simulink model "CVS Model"  (R2021a)
(part 5 of 8)

  R-Rdial Artery4 : ee_lib/Passive/Resistor  R=19.139 kOhm  R_tol=5  enable_R_tol=0  tol_distribution=1  nSigma=4  enable_operating_limits=0  operating_limit_action=2  max_working_voltage=100 V  power_rating=1 W  enable_faults=0  fault_action=1  R_faulted=inf Ohm  enable_temporal_fault=0  t_fault=1 s  enable_behavioral_fault=0  max_permissible_current=1 A  t_fail_on_current=1 s  noise_mode=0  sample_time=1e-3 s  repeatability=1  auto_seed=1105989530  user_seed=0  Tdevice=25 degC  alpha=3.93e-3 1/K  Tmeas=25 degC  thermal_mass=100 J/K  power_derating_T1=70 degC  power_derating_T2=155 degC  operating_temperature_range_vec=[-50, 150] degC  temperature_specify=off  temperature_priority=High  temperature=298.15 K  temperature_nominal_specify=off  temperature_nominal_unit=K  temperature_nominal_value=1
  R-Rdial Artery5 : ee_lib/Passive/Resistor  R=11 kOhm  R_tol=5  enable_R_tol=0  tol_distribution=1  nSigma=4  enable_operating_limits=0  operating_limit_action=2  max_working_voltage=100 V  power_rating=1 W  enable_faults=0  fault_action=1  R_faulted=inf Ohm  enable_temporal_fault=0  t_fault=1 s  enable_behavioral_fault=0  max_permissible_current=1 A  t_fail_on_current=1 s  noise_mode=0  sample_time=1e-3 s  repeatability=1  auto_seed=3610853119  user_seed=0  Tdevice=25 degC  alpha=3.93e-3 1/K  Tmeas=25 degC  thermal_mass=100 J/K  power_derating_T1=70 degC  power_derating_T2=155 degC  operating_temperature_range_vec=[-50, 150] degC  temperature_specify=off  temperature_priority=High  temperature=298.15 K  temperature_nominal_specify=off  temperature_nominal_unit=K  temperature_nominal_value=1
  R-Rdial Artery6 : ee_lib/Passive/Resistor  Commented=on  R=19.139 kOhm  R_tol=5  enable_R_tol=0  tol_distribution=1  nSigma=4  enable_operating_limits=0  operating_limit_action=2  max_working_voltage=100 V  power_rating=1 W  enable_faults=0  fault_action=1  R_faulted=inf Ohm  enable_temporal_fault=0  t_fault=1 s  enable_behavioral_fault=0  max_permissible_current=1 A  t_fail_on_current=1 s  noise_mode=0  sample_time=1e-3 s  repeatability=1  auto_seed=2563070851  user_seed=0  Tdevice=25 degC  alpha=3.93e-3 1/K  Tmeas=25 degC  thermal_mass=100 J/K  power_derating_T1=70 degC  power_derating_T2=155 degC  operating_temperature_range_vec=[-50, 150] degC  temperature_specify=off  temperature_priority=High  temperature=298.15 K  temperature_nominal_specify=off  temperature_nominal_unit=K  temperature_nominal_value=1
  R-Rdial Artery7 : ee_lib/Passive/Resistor  Commented=on  R=11 kOhm  R_tol=5  enable_R_tol=0  tol_distribution=1  nSigma=4  enable_operating_limits=0  operating_limit_action=2  max_working_voltage=100 V  power_rating=1 W  enable_faults=0  fault_action=1  R_faulted=inf Ohm  enable_temporal_fault=0  t_fault=1 s  enable_behavioral_fault=0  max_permissible_current=1 A  t_fail_on_current=1 s  noise_mode=0  sample_time=1e-3 s  repeatability=1  auto_seed=2518122460  user_seed=0  Tdevice=25 degC  alpha=3.93e-3 1/K  Tmeas=25 degC  thermal_mass=100 J/K  power_derating_T1=70 degC  power_derating_T2=155 degC  operating_temperature_range_vec=[-50, 150] degC  temperature_specify=off  temperature_priority=High  temperature=298.15 K  temperature_nominal_specify=off  temperature_nominal_unit=K  temperature_nominal_value=1
  R-Rdial Artery8 : ee_lib/Passive/Resistor  R=19.139 kOhm  R_tol=5  enable_R_tol=0  tol_distribution=1  nSigma=4  enable_operating_limits=0  operating_limit_action=2  max_working_voltage=100 V  power_rating=1 W  enable_faults=0  fault_action=1  R_faulted=inf Ohm  enable_temporal_fault=0  t_fault=1 s  enable_behavioral_fault=0  max_permissible_current=1 A  t_fail_on_current=1 s  noise_mode=0  sample_time=1e-3 s  repeatability=1  auto_seed=1105989530  user_seed=0  Tdevice=25 degC  alpha=3.93e-3 1/K  Tmeas=25 degC  thermal_mass=100 J/K  power_derating_T1=70 degC  power_derating_T2=155 degC  operating_temperature_range_vec=[-50, 150] degC  temperature_specify=off  temperature_priority=High  temperature=298.15 K  temperature_nominal_specify=off  temperature_nominal_unit=K  temperature_nominal_value=1
  R-Rdial Artery9 : ee_lib/Passive/Resistor  R=11 kOhm  R_tol=5  enable_R_tol=0  tol_distribution=1  nSigma=4  enable_operating_limits=0  operating_limit_action=2  max_working_voltage=100 V  power_rating=1 W  enable_faults=0  fault_action=1  R_faulted=inf Ohm  enable_temporal_fault=0  t_fault=1 s  enable_behavioral_fault=0  max_permissible_current=1 A  t_fail_on_current=1 s  noise_mode=0  sample_time=1e-3 s  repeatability=1  auto_seed=3610853119  user_seed=0  Tdevice=25 degC  alpha=3.93e-3 1/K  Tmeas=25 degC  thermal_mass=100 J/K  power_derating_T1=70 degC  power_derating_T2=155 degC  operating_temperature_range_vec=[-50, 150] degC  temperature_specify=off  temperature_priority=High  temperature=298.15 K  temperature_nominal_specify=off  temperature_nominal_unit=K  temperature_nominal_value=1
  R-Right Common Iliac1 : ee_lib/Passive/Resistor  Commented=on  R=0.43 kOhm  R_tol=5  enable_R_tol=0  tol_distribution=1  nSigma=4  enable_operating_limits=0  operating_limit_action=2  max_working_voltage=100 V  power_rating=1 W  enable_faults=0  fault_action=1  R_faulted=inf Ohm  enable_temporal_fault=0  t_fault=1 s  enable_behavioral_fault=0  max_permissible_current=1 A  t_fail_on_current=1 s  noise_mode=0  sample_time=1e-3 s  repeatability=1  auto_seed=1147740212  user_seed=0  Tdevice=25 degC  alpha=3.93e-3 1/K  Tmeas=25 degC  thermal_mass=100 J/K  power_derating_T1=70 degC  power_derating_T2=155 degC  operating_temperature_range_vec=[-50, 150] degC  temperature_specify=off  temperature_priority=High  temperature=298.15 K  temperature_nominal_specify=off  temperature_nominal_unit=K  temperature_nominal_value=1
  R-Right Common Iliac2 : ee_lib/Passive/Resistor  R=0.43 kOhm  R_tol=5  enable_R_tol=0  tol_distribution=1  nSigma=4  enable_operating_limits=0  operating_limit_action=2  max_working_voltage=100 V  power_rating=1 W  enable_faults=0  fault_action=1  R_faulted=inf Ohm  enable_temporal_fault=0  t_fault=1 s  enable_behavioral_fault=0  max_permissible_current=1 A  t_fail_on_current=1 s  noise_mode=0  sample_time=1e-3 s  repeatability=1  auto_seed=1092133643  user_seed=0  Tdevice=25 degC  alpha=3.93e-3 1/K  Tmeas=25 degC  thermal_mass=100 J/K  power_derating_T1=70 degC  power_derating_T2=155 degC  operating_temperature_range_vec=[-50, 150] degC  temperature_specify=off  temperature_priority=High  temperature=298.15 K  temperature_nominal_specify=off  temperature_nominal_unit=K  temperature_nominal_value=1
  R-Right Common Iliac3 : ee_lib/Passive/Resistor  Commented=on  R=0.43 kOhm  R_tol=5  enable_R_tol=0  tol_distribution=1  nSigma=4  enable_operating_limits=0  operating_limit_action=2  max_working_voltage=100 V  power_rating=1 W  enable_faults=0  fault_action=1  R_faulted=inf Ohm  enable_temporal_fault=0  t_fault=1 s  enable_behavioral_fault=0  max_permissible_current=1 A  t_fail_on_current=1 s  noise_mode=0  sample_time=1e-3 s  repeatability=1  auto_seed=4159650692  user_seed=0  Tdevice=25 degC  alpha=3.93e-3 1/K  Tmeas=25 degC  thermal_mass=100 J/K  power_derating_T1=70 degC  power_derating_T2=155 degC  operating_temperature_range_vec=[-50, 150] degC  temperature_specify=off  temperature_priority=High  temperature=298.15 K  temperature_nominal_specify=off  temperature_nominal_unit=K  temperature_nominal_value=1
  R-Right Common Iliac4 : ee_lib/Passive/Resistor  R=0.43 kOhm  R_tol=5  enable_R_tol=0  tol_distribution=1  nSigma=4  enable_operating_limits=0  operating_limit_action=2  max_working_voltage=100 V  power_rating=1 W  enable_faults=0  fault_action=1  R_faulted=inf Ohm  enable_temporal_fault=0  t_fault=1 s  enable_behavioral_fault=0  max_permissible_current=1 A  t_fail_on_current=1 s  noise_mode=0  sample_time=1e-3 s  repeatability=1  auto_seed=1092133643  user_seed=0  Tdevice=25 degC  alpha=3.93e-3 1/K  Tmeas=25 degC  thermal_mass=100 J/K  power_derating_T1=70 degC  power_derating_T2=155 degC  operating_temperature_range_vec=[-50, 150] degC  temperature_specify=off  temperature_priority=High  temperature=298.15 K  temperature_nominal_specify=off  temperature_nominal_unit=K  temperature_nominal_value=1
  R-Right External Iliac1 : ee_lib/Passive/Resistor  Commented=on  R=2.437 kOhm  R_tol=5  enable_R_tol=0  tol_distribution=1  nSigma=4  enable_operating_limits=0  operating_limit_action=2  max_working_voltage=100 V  power_rating=1 W  enable_faults=0  fault_action=1  R_faulted=inf Ohm  enable_temporal_fault=0  t_fault=1 s  enable_behavioral_fault=0  max_permissible_current=1 A  t_fail_on_current=1 s  noise_mode=0  sample_time=1e-3 s  repeatability=1  auto_seed=169678285  user_seed=0  Tdevice=25 degC  alpha=3.93e-3 1/K  Tmeas=25 degC  thermal_mass=100 J/K  power_derating_T1=70 degC  power_derating_T2=155 degC  operating_temperature_range_vec=[-50, 150] degC  temperature_specify=off  temperature_priority=High  temperature=298.15 K  temperature_nominal_specify=off  temperature_nominal_unit=K  temperature_nominal_value=1
  R-Right External Iliac2 : ee_lib/Passive/Resistor  R=2.437 kOhm  R_tol=5  enable_R_tol=0  tol_distribution=1  nSigma=4  enable_operating_limits=0  operating_limit_action=2  max_working_voltage=100 V  power_rating=1 W  enable_faults=0  fault_action=1  R_faulted=inf Ohm  enable_temporal_fault=0  t_fault=1 s  enable_behavioral_fault=0  max_permissible_current=1 A  t_fail_on_current=1 s  noise_mode=0  sample_time=1e-3 s  repeatability=1  auto_seed=3497326697  user_seed=0  Tdevice=25 degC  alpha=3.93e-3 1/K  Tmeas=25 degC  thermal_mass=100 J/K  power_derating_T1=70 degC  power_derating_T2=155 degC  operating_temperature_range_vec=[-50, 150] degC  temperature_specify=off  temperature_priority=High  temperature=298.15 K  temperature_nominal_specify=off  temperature_nominal_unit=K  temperature_nominal_value=1
  R-Right External Iliac3 : ee_lib/Passive/Resistor  Commented=on  R=2.437 kOhm  R_tol=5  enable_R_tol=0  tol_distribution=1  nSigma=4  enable_operating_limits=0  operating_limit_action=2  max_working_voltage=100 V  power_rating=1 W  enable_faults=0  fault_action=1  R_faulted=inf Ohm  enable_temporal_fault=0  t_fault=1 s  enable_behavioral_fault=0  max_permissible_current=1 A  t_fail_on_current=1 s  noise_mode=0  sample_time=1e-3 s  repeatability=1  auto_seed=2498568986  user_seed=0  Tdevice=25 degC  alpha=3.93e-3 1/K  Tmeas=25 degC  thermal_mass=100 J/K  power_derating_T1=70 degC  power_derating_T2=155 degC  operating_temperature_range_vec=[-50, 150] degC  temperature_specify=off  temperature_priority=High  temperature=298.15 K  temperature_nominal_specify=off  temperature_nominal_unit=K  temperature_nominal_value=1
  R-Right External Iliac4 : ee_lib/Passive/Resistor  R=2.437 kOhm  R_tol=5  enable_R_tol=0  tol_distribution=1  nSigma=4  enable_operating_limits=0  operating_limit_action=2  max_working_voltage=100 V  power_rating=1 W  enable_faults=0  fault_action=1  R_faulted=inf Ohm  enable_temporal_fault=0  t_fault=1 s  enable_behavioral_fault=0  max_permissible_current=1 A  t_fail_on_current=1 s  noise_mode=0  sample_time=1e-3 s  repeatability=1  auto_seed=3497326697  user_seed=0  Tdevice=25 degC  alpha=3.93e-3 1/K  Tmeas=25 degC  thermal_mass=100 J/K  power_derating_T1=70 degC  power_derating_T2=155 degC  operating_temperature_range_vec=[-50, 150] degC  temperature_specify=off  temperature_priority=High  temperature=298.15 K  temperature_nominal_specify=off  temperature_nominal_unit=K  temperature_nominal_value=1
  R-Right Femoral Artery1 : ee_lib/Passive/Resistor  Commented=on  R=2.377 kOhm  R_tol=5  enable_R_tol=0  tol_distribution=1  nSigma=4  enable_operating_limits=0  operating_limit_action=2  max_working_voltage=100 V  power_rating=1 W  enable_faults=0  fault_action=1  R_faulted=inf Ohm  enable_temporal_fault=0  t_fault=1 s  enable_behavioral_fault=0  max_permissible_current=1 A  t_fail_on_current=1 s  noise_mode=0  sample_time=1e-3 s  repeatability=1  auto_seed=1273723136  user_seed=0  Tdevice=25 degC  alpha=3.93e-3 1/K  Tmeas=25 degC  thermal_mass=100 J/K  power_derating_T1=70 degC  power_derating_T2=155 degC  operating_temperature_range_vec=[-50, 150] degC  temperature_specify=off  temperature_priority=High  temperature=298.15 K  temperature_nominal_specify=off  temperature_nominal_unit=K  temperature_nominal_value=1
  R-Right Femoral Artery2 : ee_lib/Passive/Resistor  R=2.377 kOhm  R_tol=5  enable_R_tol=0  tol_distribution=1  nSigma=4  enable_operating_limits=0  operating_limit_action=2  max_working_voltage=100 V  power_rating=1 W  enable_faults=0  fault_action=1  R_faulted=inf Ohm  enable_temporal_fault=0  t_fault=1 s  enable_behavioral_fault=0  max_permissible_current=1 A  t_fail_on_current=1 s  noise_mode=0  sample_time=1e-3 s  repeatability=1  auto_seed=1045931777  user_seed=0  Tdevice=25 degC  alpha=3.93e-3 1/K  Tmeas=25 degC  thermal_mass=100 J/K  power_derating_T1=70 degC  power_derating_T2=155 degC  operating_temperature_range_vec=[-50, 150] degC  temperature_specify=off  temperature_priority=High  temperature=298.15 K  temperature_nominal_specify=off  temperature_nominal_unit=K  temperature_nominal_value=1
  R-Right Femoral Artery3 : ee_lib/Passive/Resistor  Commented=on  R=2.377 kOhm  R_tol=5  enable_R_tol=0  tol_distribution=1  nSigma=4  enable_operating_limits=0  operating_limit_action=2  max_working_voltage=100 V  power_rating=1 W  enable_faults=0  fault_action=1  R_faulted=inf Ohm  enable_temporal_fault=0  t_fault=1 s  enable_behavioral_fault=0  max_permissible_current=1 A  t_fail_on_current=1 s  noise_mode=0  sample_time=1e-3 s  repeatability=1  auto_seed=428638988  user_seed=0  Tdevice=25 degC  alpha=3.93e-3 1/K  Tmeas=25 degC  thermal_mass=100 J/K  power_derating_T1=70 degC  power_derating_T2=155 degC  operating_temperature_range_vec=[-50, 150] degC  temperature_specify=off  temperature_priority=High  temperature=298.15 K  temperature_nominal_specify=off  temperature_nominal_unit=K  temperature_nominal_value=1
  R-Right Femoral Artery4 : ee_lib/Passive/Resistor  R=2.377 kOhm  R_tol=5  enable_R_tol=0  tol_distribution=1  nSigma=4  enable_operating_limits=0  operating_limit_action=2  max_working_voltage=100 V  power_rating=1 W  enable_faults=0  fault_action=1  R_faulted=inf Ohm  enable_temporal_fault=0  t_fault=1 s  enable_behavioral_fault=0  max_permissible_current=1 A  t_fail_on_current=1 s  noise_mode=0  sample_time=1e-3 s  repeatability=1  auto_seed=1045931777  user_seed=0  Tdevice=25 degC  alpha=3.93e-3 1/K  Tmeas=25 degC  thermal_mass=100 J/K  power_derating_T1=70 degC  power_derating_T2=155 degC  operating_temperature_range_vec=[-50, 150] degC  temperature_specify=off  temperature_priority=High  temperature=298.15 K  temperature_nominal_specify=off  temperature_nominal_unit=K  temperature_nominal_value=1
  R-Right Pulmonary Artery1 : ee_lib/Passive/Resistor  Commented=on  R=4 kOhm  R_tol=5  enable_R_tol=0  tol_distribution=1  nSigma=4  enable_operating_limits=0  operating_limit_action=2  max_working_voltage=100 V  power_rating=1 W  enable_faults=0  fault_action=1  R_faulted=inf Ohm  enable_temporal_fault=0  t_fault=1 s  enable_behavioral_fault=0  max_permissible_current=1 A  t_fail_on_current=1 s  noise_mode=0  sample_time=1e-3 s  repeatability=1  auto_seed=2389569373  user_seed=0  Tdevice=25 degC  alpha=3.93e-3 1/K  Tmeas=25 degC  thermal_mass=100 J/K  power_derating_T1=70 degC  power_derating_T2=155 degC  operating_temperature_range_vec=[-50, 150] degC  temperature_specify=off  temperature_priority=High  temperature=298.15 K  temperature_nominal_specify=off  temperature_nominal_unit=K  temperature_nominal_value=1
  R-Right Pulmonary Artery2 : ee_lib/Passive/Resistor  R=4 kOhm  R_tol=5  enable_R_tol=0  tol_distribution=1  nSigma=4  enable_operating_limits=0  operating_limit_action=2  max_working_voltage=100 V  power_rating=1 W  enable_faults=0  fault_action=1  R_faulted=inf Ohm  enable_temporal_fault=0  t_fault=1 s  enable_behavioral_fault=0  max_permissible_current=1 A  t_fail_on_current=1 s  noise_mode=0  sample_time=1e-3 s  repeatability=1  auto_seed=3991156871  user_seed=0  Tdevice=25 degC  alpha=3.93e-3 1/K  Tmeas=25 degC  thermal_mass=100 J/K  power_derating_T1=70 degC  power_derating_T2=155 degC  operating_temperature_range_vec=[-50, 150] degC  temperature_specify=off  temperature_priority=High  temperature=298.15 K  temperature_nominal_specify=off  temperature_nominal_unit=K  temperature_nominal_value=1
  R-Right Pulmonary Artery3 : ee_lib/Passive/Resistor  Commented=on  R=4 kOhm  R_tol=5  enable_R_tol=0  tol_distribution=1  nSigma=4  enable_operating_limits=0  operating_limit_action=2  max_working_voltage=100 V  power_rating=1 W  enable_faults=0  fault_action=1  R_faulted=inf Ohm  enable_temporal_fault=0  t_fault=1 s  enable_behavioral_fault=0  max_permissible_current=1 A  t_fail_on_current=1 s  noise_mode=0  sample_time=1e-3 s  repeatability=1  auto_seed=715553671  user_seed=0  Tdevice=25 degC  alpha=3.93e-3 1/K  Tmeas=25 degC  thermal_mass=100 J/K  power_derating_T1=70 degC  power_derating_T2=155 degC  operating_temperature_range_vec=[-50, 150] degC  temperature_specify=off  temperature_priority=High  temperature=298.15 K  temperature_nominal_specify=off  temperature_nominal_unit=K  temperature_nominal_value=1
  R-Right Pulmonary Artery4 : ee_lib/Passive/Resistor  R=4 kOhm  R_tol=5  enable_R_tol=0  tol_distribution=1  nSigma=4  enable_operating_limits=0  operating_limit_action=2  max_working_voltage=100 V  power_rating=1 W  enable_faults=0  fault_action=1  R_faulted=inf Ohm  enable_temporal_fault=0  t_fault=1 s  enable_behavioral_fault=0  max_permissible_current=1 A  t_fail_on_current=1 s  noise_mode=0  sample_time=1e-3 s  repeatability=1  auto_seed=3991156871  user_seed=0  Tdevice=25 degC  alpha=3.93e-3 1/K  Tmeas=25 degC  thermal_mass=100 J/K  power_derating_T1=70 degC  power_derating_T2=155 degC  operating_temperature_range_vec=[-50, 150] degC  temperature_specify=off  temperature_priority=High  temperature=298.15 K  temperature_nominal_specify=off  temperature_nominal_unit=K  temperature_nominal_value=1
  R-Ulnar Artery2 : ee_lib/Passive/Resistor  Commented=on  R=7.63 kOhm  R_tol=5  enable_R_tol=0  tol_distribution=1  nSigma=4  enable_operating_limits=0  operating_limit_action=2  max_working_voltage=100 V  power_rating=1 W  enable_faults=0  fault_action=1  R_faulted=inf Ohm  enable_temporal_fault=0  t_fault=1 s  enable_behavioral_fault=0  max_permissible_current=1 A  t_fail_on_current=1 s  noise_mode=0  sample_time=1e-3 s  repeatability=1  auto_seed=4162143160  user_seed=0  Tdevice=25 degC  alpha=3.93e-3 1/K  Tmeas=25 degC  thermal_mass=100 J/K  power_derating_T1=70 degC  power_derating_T2=155 degC  operating_temperature_range_vec=[-50, 150] degC  temperature_specify=off  temperature_priority=High  temperature=298.15 K  temperature_nominal_specify=off  temperature_nominal_unit=K  temperature_nominal_value=1
  R-Ulnar Artery3 : ee_lib/Passive/Resistor  Commented=on  R=4.4 kOhm  R_tol=5  enable_R_tol=0  tol_distribution=1  nSigma=4  enable_operating_limits=0  operating_limit_action=2  max_working_voltage=100 V  power_rating=1 W  enable_faults=0  fault_action=1  R_faulted=inf Ohm  enable_temporal_fault=0  t_fault=1 s  enable_behavioral_fault=0  max_permissible_current=1 A  t_fail_on_current=1 s  noise_mode=0  sample_time=1e-3 s  repeatability=1  auto_seed=2959768097  user_seed=0  Tdevice=25 degC  alpha=3.93e-3 1/K  Tmeas=25 degC  thermal_mass=100 J/K  power_derating_T1=70 degC  power_derating_T2=155 degC  operating_temperature_range_vec=[-50, 150] degC  temperature_specify=off  temperature_priority=High  temperature=298.15 K  temperature_nominal_specify=off  temperature_nominal_unit=K  temperature_nominal_value=1
  R-Ulnar Artery4 : ee_lib/Passive/Resistor  R=7.63 kOhm  R_tol=5  enable_R_tol=0  tol_distribution=1  nSigma=4  enable_operating_limits=0  operating_limit_action=2  max_working_voltage=100 V  power_rating=1 W  enable_faults=0  fault_action=1  R_faulted=inf Ohm  enable_temporal_fault=0  t_fault=1 s  enable_behavioral_fault=0  max_permissible_current=1 A  t_fail_on_current=1 s  noise_mode=0  sample_time=1e-3 s  repeatability=1  auto_seed=1503168829  user_seed=0  Tdevice=25 degC  alpha=3.93e-3 1/K  Tmeas=25 degC  thermal_mass=100 J/K  power_derating_T1=70 degC  power_derating_T2=155 degC  operating_temperature_range_vec=[-50, 150] degC  temperature_specify=off  temperature_priority=High  temperature=298.15 K  temperature_nominal_specify=off  temperature_nominal_unit=K  temperature_nominal_value=1
  R-Ulnar Artery5 : ee_lib/Passive/Resistor  R=4.4 kOhm  R_tol=5  enable_R_tol=0  tol_distribution=1  nSigma=4  enable_operating_limits=0  operating_limit_action=2  max_working_voltage=100 V  power_rating=1 W  enable_faults=0  fault_action=1  R_faulted=inf Ohm  enable_temporal_fault=0  t_fault=1 s  enable_behavioral_fault=0  max_permissible_current=1 A  t_fail_on_current=1 s  noise_mode=0  sample_time=1e-3 s  repeatability=1  auto_seed=844370171  user_seed=0  Tdevice=25 degC  alpha=3.93e-3 1/K  Tmeas=25 degC  thermal_mass=100 J/K  power_derating_T1=70 degC  power_derating_T2=155 degC  operating_temperature_range_vec=[-50, 150] degC  temperature_specify=off  temperature_priority=High  temperature=298.15 K  temperature_nominal_specify=off  temperature_nominal_unit=K  temperature_nominal_value=1
  R-Ulnar Artery6 : ee_lib/Passive/Resistor  Commented=on  R=7.63 kOhm  R_tol=5  enable_R_tol=0  tol_distribution=1  nSigma=4  enable_operating_limits=0  operating_limit_action=2  max_working_voltage=100 V  power_rating=1 W  enable_faults=0  fault_action=1  R_faulted=inf Ohm  enable_temporal_fault=0  t_fault=1 s  enable_behavioral_fault=0  max_permissible_current=1 A  t_fail_on_current=1 s  noise_mode=0  sample_time=1e-3 s  repeatability=1  auto_seed=438489510  user_seed=0  Tdevice=25 degC  alpha=3.93e-3 1/K  Tmeas=25 degC  thermal_mass=100 J/K  power_derating_T1=70 degC  power_derating_T2=155 degC  operating_temperature_range_vec=[-50, 150] degC  temperature_specify=off  temperature_priority=High  temperature=298.15 K  temperature_nominal_specify=off  temperature_nominal_unit=K  temperature_nominal_value=1
  R-Ulnar Artery7 : ee_lib/Passive/Resistor  Commented=on  R=4.4 kOhm  R_tol=5  enable_R_tol=0  tol_distribution=1  nSigma=4  enable_operating_limits=0  operating_limit_action=2  max_working_voltage=100 V  power_rating=1 W  enable_faults=0  fault_action=1  R_faulted=inf Ohm  enable_temporal_fault=0  t_fault=1 s  enable_behavioral_fault=0  max_permissible_current=1 A  t_fail_on_current=1 s  noise_mode=0  sample_time=1e-3 s  repeatability=1  auto_seed=628126532  user_seed=0  Tdevice=25 degC  alpha=3.93e-3 1/K  Tmeas=25 degC  thermal_mass=100 J/K  power_derating_T1=70 degC  power_derating_T2=155 degC  operating_temperature_range_vec=[-50, 150] degC  temperature_specify=off  temperature_priority=High  temperature=298.15 K  temperature_nominal_specify=off  temperature_nominal_unit=K  temperature_nominal_value=1
  R-Ulnar Artery8 : ee_lib/Passive/Resistor  R=7.63 kOhm  R_tol=5  enable_R_tol=0  tol_distribution=1  nSigma=4  enable_operating_limits=0  operating_limit_action=2  max_working_voltage=100 V  power_rating=1 W  enable_faults=0  fault_action=1  R_faulted=inf Ohm  enable_temporal_fault=0  t_fault=1 s  enable_behavioral_fault=0  max_permissible_current=1 A  t_fail_on_current=1 s  noise_mode=0  sample_time=1e-3 s  repeatability=1  auto_seed=1503168829  user_seed=0  Tdevice=25 degC  alpha=3.93e-3 1/K  Tmeas=25 degC  thermal_mass=100 J/K  power_derating_T1=70 degC  power_derating_T2=155 degC  operating_temperature_range_vec=[-50, 150] degC  temperature_specify=off  temperature_priority=High  temperature=298.15 K  temperature_nominal_specify=off  temperature_nominal_unit=K  temperature_nominal_value=1
  R-Ulnar Artery9 : ee_lib/Passive/Resistor  R=4.4 kOhm  R_tol=5  enable_R_tol=0  tol_distribution=1  nSigma=4  enable_operating_limits=0  operating_limit_action=2  max_working_voltage=100 V  power_rating=1 W  enable_faults=0  fault_action=1  R_faulted=inf Ohm  enable_temporal_fault=0  t_fault=1 s  enable_behavioral_fault=0  max_permissible_current=1 A  t_fail_on_current=1 s  noise_mode=0  sample_time=1e-3 s  repeatability=1  auto_seed=844370171  user_seed=0  Tdevice=25 degC  alpha=3.93e-3 1/K  Tmeas=25 degC  thermal_mass=100 J/K  power_derating_T1=70 degC  power_derating_T2=155 degC  operating_temperature_range_vec=[-50, 150] degC  temperature_specify=off  temperature_priority=High  temperature=298.15 K  temperature_nominal_specify=off  temperature_nominal_unit=K  temperature_nominal_value=1
  R-Visco AT1 : ee_lib/Passive/Resistor  Commented=on  R=0.005 kOhm  R_tol=5  enable_R_tol=0  tol_distribution=1  nSigma=4  enable_operating_limits=0  operating_limit_action=2  max_working_voltage=100 V  power_rating=1 W  enable_faults=0  fault_action=1  R_faulted=inf Ohm  enable_temporal_fault=0  t_fault=1 s  enable_behavioral_fault=0  max_permissible_current=1 A  t_fail_on_current=1 s  noise_mode=0  sample_time=1e-3 s  repeatability=1  auto_seed=3083277128  user_seed=0  Tdevice=25 degC  alpha=3.93e-3 1/K  Tmeas=25 degC  thermal_mass=100 J/K  power_derating_T1=70 degC  power_derating_T2=155 degC  operating_temperature_range_vec=[-50, 150] degC  temperature_specify=off  temperature_priority=High  temperature=298.15 K  temperature_nominal_specify=off  temperature_nominal_unit=K  temperature_nominal_value=1
  R-Visco AT2 : ee_lib/Passive/Resistor  R=0.005 kOhm  R_tol=5  enable_R_tol=0  tol_distribution=1  nSigma=4  enable_operating_limits=0  operating_limit_action=2  max_working_voltage=100 V  power_rating=1 W  enable_faults=0  fault_action=1  R_faulted=inf Ohm  enable_temporal_fault=0  t_fault=1 s  enable_behavioral_fault=0  max_permissible_current=1 A  t_fail_on_current=1 s  noise_mode=0  sample_time=1e-3 s  repeatability=1  auto_seed=1078396959  user_seed=0  Tdevice=25 degC  alpha=3.93e-3 1/K  Tmeas=25 degC  thermal_mass=100 J/K  power_derating_T1=70 degC  power_derating_T2=155 degC  operating_temperature_range_vec=[-50, 150] degC  temperature_specify=off  temperature_priority=High  temperature=298.15 K  temperature_nominal_specify=off  temperature_nominal_unit=K  temperature_nominal_value=1
  R-Visco AT3 : ee_lib/Passive/Resistor  Commented=on  R=0.005 kOhm  R_tol=5  enable_R_tol=0  tol_distribution=1  nSigma=4  enable_operating_limits=0  operating_limit_action=2  max_working_voltage=100 V  power_rating=1 W  enable_faults=0  fault_action=1  R_faulted=inf Ohm  enable_temporal_fault=0  t_fault=1 s  enable_behavioral_fault=0  max_permissible_current=1 A  t_fail_on_current=1 s  noise_mode=0  sample_time=1e-3 s  repeatability=1  auto_seed=2884348711  user_seed=0  Tdevice=25 degC  alpha=3.93e-3 1/K  Tmeas=25 degC  thermal_mass=100 J/K  power_derating_T1=70 degC  power_derating_T2=155 degC  operating_temperature_range_vec=[-50, 150] degC  temperature_specify=off  temperature_priority=High  temperature=298.15 K  temperature_nominal_specify=off  temperature_nominal_unit=K  temperature_nominal_value=1
  R-Visco AT4 : ee_lib/Passive/Resistor  R=0.005 kOhm  R_tol=5  enable_R_tol=0  tol_distribution=1  nSigma=4  enable_operating_limits=0  operating_limit_action=2  max_working_voltage=100 V  power_rating=1 W  enable_faults=0  fault_action=1  R_faulted=inf Ohm  enable_temporal_fault=0  t_fault=1 s  enable_behavioral_fault=0  max_permissible_current=1 A  t_fail_on_current=1 s  noise_mode=0  sample_time=1e-3 s  repeatability=1  auto_seed=1078396959  user_seed=0  Tdevice=25 degC  alpha=3.93e-3 1/K  Tmeas=25 degC  thermal_mass=100 J/K  power_derating_T1=70 degC  power_derating_T2=155 degC  operating_temperature_range_vec=[-50, 150] degC  temperature_specify=off  temperature_priority=High  temperature=298.15 K  temperature_nominal_specify=off  temperature_nominal_unit=K  temperature_nominal_value=1
  R-Visco Hepatic 1 : ee_lib/Passive/Resistor  Commented=on  R=0.005 kOhm  R_tol=5  enable_R_tol=0  tol_distribution=1  nSigma=4  enable_operating_limits=0  operating_limit_action=2  max_working_voltage=100 V  power_rating=1 W  enable_faults=0  fault_action=1  R_faulted=inf Ohm  enable_temporal_fault=0  t_fault=1 s  enable_behavioral_fault=0  max_permissible_current=1 A  t_fail_on_current=1 s  noise_mode=0  sample_time=1e-3 s  repeatability=1  auto_seed=2401011786  user_seed=0  Tdevice=25 degC  alpha=3.93e-3 1/K  Tmeas=25 degC  thermal_mass=100 J/K  power_derating_T1=70 degC  power_derating_T2=155 degC  operating_temperature_range_vec=[-50, 150] degC  temperature_specify=off  temperature_priority=High  temperature=298.15 K  temperature_nominal_specify=off  temperature_nominal_unit=K  temperature_nominal_value=1
  R-Visco Hepatic 2 : ee_lib/Passive/Resistor  R=0.005 kOhm  R_tol=5  enable_R_tol=0  tol_distribution=1  nSigma=4  enable_operating_limits=0  operating_limit_action=2  max_working_voltage=100 V  power_rating=1 W  enable_faults=0  fault_action=1  R_faulted=inf Ohm  enable_temporal_fault=0  t_fault=1 s  enable_behavioral_fault=0  max_permissible_current=1 A  t_fail_on_current=1 s  noise_mode=0  sample_time=1e-3 s  repeatability=1  auto_seed=2645891737  user_seed=0  Tdevice=25 degC  alpha=3.93e-3 1/K  Tmeas=25 degC  thermal_mass=100 J/K  power_derating_T1=70 degC  power_derating_T2=155 degC  operating_temperature_range_vec=[-50, 150] degC  temperature_specify=off  temperature_priority=High  temperature=298.15 K  temperature_nominal_specify=off  temperature_nominal_unit=K  temperature_nominal_value=1
  R-Visco Hepatic 3 : ee_lib/Passive/Resistor  Commented=on  R=0.005 kOhm  R_tol=5  enable_R_tol=0  tol_distribution=1  nSigma=4  enable_operating_limits=0  operating_limit_action=2  max_working_voltage=100 V  power_rating=1 W  enable_faults=0  fault_action=1  R_faulted=inf Ohm  enable_temporal_fault=0  t_fault=1 s  enable_behavioral_fault=0  max_permissible_current=1 A  t_fail_on_current=1 s  noise_mode=0  sample_time=1e-3 s  repeatability=1  auto_seed=2748148490  user_seed=0  Tdevice=25 degC  alpha=3.93e-3 1/K  Tmeas=25 degC  thermal_mass=100 J/K  power_derating_T1=70 degC  power_derating_T2=155 degC  operating_temperature_range_vec=[-50, 150] degC  temperature_specify=off  temperature_priority=High  temperature=298.15 K  temperature_nominal_specify=off  temperature_nominal_unit=K  temperature_nominal_value=1
  R-Visco Hepatic 4 : ee_lib/Passive/Resistor  R=0.005 kOhm  R_tol=5  enable_R_tol=0  tol_distribution=1  nSigma=4  enable_operating_limits=0  operating_limit_action=2  max_working_voltage=100 V  power_rating=1 W  enable_faults=0  fault_action=1  R_faulted=inf Ohm  enable_temporal_fault=0  t_fault=1 s  enable_behavioral_fault=0  max_permissible_current=1 A  t_fail_on_current=1 s  noise_mode=0  sample_time=1e-3 s  repeatability=1  auto_seed=2645891737  user_seed=0  Tdevice=25 degC  alpha=3.93e-3 1/K  Tmeas=25 degC  thermal_mass=100 J/K  power_derating_T1=70 degC  power_derating_T2=155 degC  operating_temperature_range_vec=[-50, 150] degC  temperature_specify=off  temperature_priority=High  temperature=298.15 K  temperature_nominal_specify=off  temperature_nominal_unit=K  temperature_nominal_value=1
  R-Visco IM1 : ee_lib/Passive/Resistor  Commented=on  R=0.05 kOhm  R_tol=5  enable_R_tol=0  tol_distribution=1  nSigma=4  enable_operating_limits=0  operating_limit_action=2  max_working_voltage=100 V  power_rating=1 W  enable_faults=0  fault_action=1  R_faulted=inf Ohm  enable_temporal_fault=0  t_fault=1 s  enable_behavioral_fault=0  max_permissible_current=1 A  t_fail_on_current=1 s  noise_mode=0  sample_time=1e-3 s  repeatability=1  auto_seed=2290738880  user_seed=0  Tdevice=25 degC  alpha=3.93e-3 1/K  Tmeas=25 degC  thermal_mass=100 J/K  power_derating_T1=70 degC  power_derating_T2=155 degC  operating_temperature_range_vec=[-50, 150] degC  temperature_specify=off  temperature_priority=High  temperature=298.15 K  temperature_nominal_specify=off  temperature_nominal_unit=K  temperature_nominal_value=1
  R-Visco IM2 : ee_lib/Passive/Resistor  R=0.05 kOhm  R_tol=5  enable_R_tol=0  tol_distribution=1  nSigma=4  enable_operating_limits=0  operating_limit_action=2  max_working_voltage=100 V  power_rating=1 W  enable_faults=0  fault_action=1  R_faulted=inf Ohm  enable_temporal_fault=0  t_fault=1 s  enable_behavioral_fault=0  max_permissible_current=1 A  t_fail_on_current=1 s  noise_mode=0  sample_time=1e-3 s  repeatability=1  auto_seed=2032760128  user_seed=0  Tdevice=25 degC  alpha=3.93e-3 1/K  Tmeas=25 degC  thermal_mass=100 J/K  power_derating_T1=70 degC  power_derating_T2=155 degC  operating_temperature_range_vec=[-50, 150] degC  temperature_specify=off  temperature_priority=High  temperature=298.15 K  temperature_nominal_specify=off  temperature_nominal_unit=K  temperature_nominal_value=1
  R-Visco IM3 : ee_lib/Passive/Resistor  Commented=on  R=0.05 kOhm  R_tol=5  enable_R_tol=0  tol_distribution=1  nSigma=4  enable_operating_limits=0  operating_limit_action=2  max_working_voltage=100 V  power_rating=1 W  enable_faults=0  fault_action=1  R_faulted=inf Ohm  enable_temporal_fault=0  t_fault=1 s  enable_behavioral_fault=0  max_permissible_current=1 A  t_fail_on_current=1 s  noise_mode=0  sample_time=1e-3 s  repeatability=1  auto_seed=1599598085  user_seed=0  Tdevice=25 degC  alpha=3.93e-3 1/K  Tmeas=25 degC  thermal_mass=100 J/K  power_derating_T1=70 degC  power_derating_T2=155 degC  operating_temperature_range_vec=[-50, 150] degC  temperature_specify=off  temperature_priority=High  temperature=298.15 K  temperature_nominal_specify=off  temperature_nominal_unit=K  temperature_nominal_value=1
  R-Visco IM4 : ee_lib/Passive/Resistor  R=0.05 kOhm  R_tol=5  enable_R_tol=0  tol_distribution=1  nSigma=4  enable_operating_limits=0  operating_limit_action=2  max_working_voltage=100 V  power_rating=1 W  enable_faults=0  fault_action=1  R_faulted=inf Ohm  enable_temporal_fault=0  t_fault=1 s  enable_behavioral_fault=0  max_permissible_current=1 A  t_fail_on_current=1 s  noise_mode=0  sample_time=1e-3 s  repeatability=1  auto_seed=2032760128  user_seed=0  Tdevice=25 degC  alpha=3.93e-3 1/K  Tmeas=25 degC  thermal_mass=100 J/K  power_derating_T1=70 degC  power_derating_T2=155 degC  operating_temperature_range_vec=[-50, 150] degC  temperature_specify=off  temperature_priority=High  temperature=298.15 K  temperature_nominal_specify=off  temperature_nominal_unit=K  temperature_nominal_value=1
  R-Visco LCI1 : ee_lib/Passive/Resistor  Commented=on  R=0.005 kOhm  R_tol=5  enable_R_tol=0  tol_distribution=1  nSigma=4  enable_operating_limits=0  operating_limit_action=2  max_working_voltage=100 V  power_rating=1 W  enable_faults=0  fault_action=1  R_faulted=inf Ohm  enable_temporal_fault=0  t_fault=1 s  enable_behavioral_fault=0  max_permissible_current=1 A  t_fail_on_current=1 s  noise_mode=0  sample_time=1e-3 s  repeatability=1  auto_seed=3761205951  user_seed=0  Tdevice=25 degC  alpha=3.93e-3 1/K  Tmeas=25 degC  thermal_mass=100 J/K  power_derating_T1=70 degC  power_derating_T2=155 degC  operating_temperature_range_vec=[-50, 150] degC  temperature_specify=off  temperature_priority=High  temperature=298.15 K  temperature_nominal_specify=off  temperature_nominal_unit=K  temperature_nominal_value=1
  R-Visco LCI2 : ee_lib/Passive/Resistor  R=0.005 kOhm  R_tol=5  enable_R_tol=0  tol_distribution=1  nSigma=4  enable_operating_limits=0  operating_limit_action=2  max_working_voltage=100 V  power_rating=1 W  enable_faults=0  fault_action=1  R_faulted=inf Ohm  enable_temporal_fault=0  t_fault=1 s  enable_behavioral_fault=0  max_permissible_current=1 A  t_fail_on_current=1 s  noise_mode=0  sample_time=1e-3 s  repeatability=1  auto_seed=1510366082  user_seed=0  Tdevice=25 degC  alpha=3.93e-3 1/K  Tmeas=25 degC  thermal_mass=100 J/K  power_derating_T1=70 degC  power_derating_T2=155 degC  operating_temperature_range_vec=[-50, 150] degC  temperature_specify=off  temperature_priority=High  temperature=298.15 K  temperature_nominal_specify=off  temperature_nominal_unit=K  temperature_nominal_value=1
  R-Visco LCI3 : ee_lib/Passive/Resistor  Commented=on  R=0.005 kOhm  R_tol=5  enable_R_tol=0  tol_distribution=1  nSigma=4  enable_operating_limits=0  operating_limit_action=2  max_working_voltage=100 V  power_rating=1 W  enable_faults=0  fault_action=1  R_faulted=inf Ohm  enable_temporal_fault=0  t_fault=1 s  enable_behavioral_fault=0  max_permissible_current=1 A  t_fail_on_current=1 s  noise_mode=0  sample_time=1e-3 s  repeatability=1  auto_seed=699534063  user_seed=0  Tdevice=25 degC  alpha=3.93e-3 1/K  Tmeas=25 degC  thermal_mass=100 J/K  power_derating_T1=70 degC  power_derating_T2=155 degC  operating_temperature_range_vec=[-50, 150] degC  temperature_specify=off  temperature_priority=High  temperature=298.15 K  temperature_nominal_specify=off  temperature_nominal_unit=K  temperature_nominal_value=1
  R-Visco LCI4 : ee_lib/Passive/Resistor  R=0.005 kOhm  R_tol=5  enable_R_tol=0  tol_distribution=1  nSigma=4  enable_operating_limits=0  operating_limit_action=2  max_working_voltage=100 V  power_rating=1 W  enable_faults=0  fault_action=1  R_faulted=inf Ohm  enable_temporal_fault=0  t_fault=1 s  enable_behavioral_fault=0  max_permissible_current=1 A  t_fail_on_current=1 s  noise_mode=0  sample_time=1e-3 s  repeatability=1  auto_seed=1510366082  user_seed=0  Tdevice=25 degC  alpha=3.93e-3 1/K  Tmeas=25 degC  thermal_mass=100 J/K  power_derating_T1=70 degC  power_derating_T2=155 degC  operating_temperature_range_vec=[-50, 150] degC  temperature_specify=off  temperature_priority=High  temperature=298.15 K  temperature_nominal_specify=off  temperature_nominal_unit=K  temperature_nominal_value=1
  R-Visco LEI1 : ee_lib/Passive/Resistor  Commented=on  R=0.005 kOhm  R_tol=5  enable_R_tol=0  tol_distribution=1  nSigma=4  enable_operating_limits=0  operating_limit_action=2  max_working_voltage=100 V  power_rating=1 W  enable_faults=0  fault_action=1  R_faulted=inf Ohm  enable_temporal_fault=0  t_fault=1 s  enable_behavioral_fault=0  max_permissible_current=1 A  t_fail_on_current=1 s  noise_mode=0  sample_time=1e-3 s  repeatability=1  auto_seed=1688345600  user_seed=0  Tdevice=25 degC  alpha=3.93e-3 1/K  Tmeas=25 degC  thermal_mass=100 J/K  power_derating_T1=70 degC  power_derating_T2=155 degC  operating_temperature_range_vec=[-50, 150] degC  temperature_specify=off  temperature_priority=High  temperature=298.15 K  temperature_nominal_specify=off  temperature_nominal_unit=K  temperature_nominal_value=1
  R-Visco LEI2 : ee_lib/Passive/Resistor  R=0.005 kOhm  R_tol=5  enable_R_tol=0  tol_distribution=1  nSigma=4  enable_operating_limits=0  operating_limit_action=2  max_working_voltage=100 V  power_rating=1 W  enable_faults=0  fault_action=1  R_faulted=inf Ohm  enable_temporal_fault=0  t_fault=1 s  enable_behavioral_fault=0  max_permissible_current=1 A  t_fail_on_current=1 s  noise_mode=0  sample_time=1e-3 s  repeatability=1  auto_seed=3568381785  user_seed=0  Tdevice=25 degC  alpha=3.93e-3 1/K  Tmeas=25 degC  thermal_mass=100 J/K  power_derating_T1=70 degC  power_derating_T2=155 degC  operating_temperature_range_vec=[-50, 150] degC  temperature_specify=off  temperature_priority=High  temperature=298.15 K  temperature_nominal_specify=off  temperature_nominal_unit=K  temperature_nominal_value=1
  R-Visco LEI3 : ee_lib/Passive/Resistor  Commented=on  R=0.005 kOhm  R_tol=5  enable_R_tol=0  tol_distribution=1  nSigma=4  enable_operating_limits=0  operating_limit_action=2  max_working_voltage=100 V  power_rating=1 W  enable_faults=0  fault_action=1  R_faulted=inf Ohm  enable_temporal_fault=0  t_fault=1 s  enable_behavioral_fault=0  max_permissible_current=1 A  t_fail_on_current=1 s  noise_mode=0  sample_time=1e-3 s  repeatability=1  auto_seed=1672970543  user_seed=0  Tdevice=25 degC  alpha=3.93e-3 1/K  Tmeas=25 degC  thermal_mass=100 J/K  power_derating_T1=70 degC  power_derating_T2=155 degC  operating_temperature_range_vec=[-50, 150] degC  temperature_specify=off  temperature_priority=High  temperature=298.15 K  temperature_nominal_specify=off  temperature_nominal_unit=K  temperature_nominal_value=1
  R-Visco LEI4 : ee_lib/Passive/Resistor  R=0.005 kOhm  R_tol=5  enable_R_tol=0  tol_distribution=1  nSigma=4  enable_operating_limits=0  operating_limit_action=2  max_working_voltage=100 V  power_rating=1 W  enable_faults=0  fault_action=1  R_faulted=inf Ohm  enable_temporal_fault=0  t_fault=1 s  enable_behavioral_fault=0  max_permissible_current=1 A  t_fail_on_current=1 s  noise_mode=0  sample_time=1e-3 s  repeatability=1  auto_seed=3568381785  user_seed=0  Tdevice=25 degC  alpha=3.93e-3 1/K  Tmeas=25 degC  thermal_mass=100 J/K  power_derating_T1=70 degC  power_derating_T2=155 degC  operating_temperature_range_vec=[-50, 150] degC  temperature_specify=off  temperature_priority=High  temperature=298.15 K  temperature_nominal_specify=off  temperature_nominal_unit=K  temperature_nominal_value=1
  R-Visco LFA1 : ee_lib/Passive/Resistor  Commented=on  R=0.005 kOhm  R_tol=5  enable_R_tol=0  tol_distribution=1  nSigma=4  enable_operating_limits=0  operating_limit_action=2  max_working_voltage=100 V  power_rating=1 W  enable_faults=0  fault_action=1  R_faulted=inf Ohm  enable_temporal_fault=0  t_fault=1 s  enable_behavioral_fault=0  max_permissible_current=1 A  t_fail_on_current=1 s  noise_mode=0  sample_time=1e-3 s  repeatability=1  auto_seed=1967382518  user_seed=0  Tdevice=25 degC  alpha=3.93e-3 1/K  Tmeas=25 degC  thermal_mass=100 J/K  power_derating_T1=70 degC  power_derating_T2=155 degC  operating_temperature_range_vec=[-50, 150] degC  temperature_specify=off  temperature_priority=High  temperature=298.15 K  temperature_nominal_specify=off  temperature_nominal_unit=K  temperature_nominal_value=1
  R-Visco LFA2 : ee_lib/Passive/Resistor  R=0.005 kOhm  R_tol=5  enable_R_tol=0  tol_distribution=1  nSigma=4  enable_operating_limits=0  operating_limit_action=2  max_working_voltage=100 V  power_rating=1 W  enable_faults=0  fault_action=1  R_faulted=inf Ohm  enable_temporal_fault=0  t_fault=1 s  enable_behavioral_fault=0  max_permissible_current=1 A  t_fail_on_current=1 s  noise_mode=0  sample_time=1e-3 s  repeatability=1  auto_seed=2513690131  user_seed=0  Tdevice=25 degC  alpha=3.93e-3 1/K  Tmeas=25 degC  thermal_mass=100 J/K  power_derating_T1=70 degC  power_derating_T2=155 degC  operating_temperature_range_vec=[-50, 150] degC  temperature_specify=off  temperature_priority=High  temperature=298.15 K  temperature_nominal_specify=off  temperature_nominal_unit=K  temperature_nominal_value=1
  R-Visco LFA3 : ee_lib/Passive/Resistor  Commented=on  R=0.005 kOhm  R_tol=5  enable_R_tol=0  tol_distribution=1  nSigma=4  enable_operating_limits=0  operating_limit_action=2  max_working_voltage=100 V  power_rating=1 W  enable_faults=0  fault_action=1  R_faulted=inf Ohm  enable_temporal_fault=0  t_fault=1 s  enable_behavioral_fault=0  max_permissible_current=1 A  t_fail_on_current=1 s  noise_mode=0  sample_time=1e-3 s  repeatability=1  auto_seed=3435873190  user_seed=0  Tdevice=25 degC  alpha=3.93e-3 1/K  Tmeas=25 degC  thermal_mass=100 J/K  power_derating_T1=70 degC  power_derating_T2=155 degC  operating_temperature_range_vec=[-50, 150] degC  temperature_specify=off  temperature_priority=High  temperature=298.15 K  temperature_nominal_specify=off  temperature_nominal_unit=K  temperature_nominal_value=1
  R-Visco LFA4 : ee_lib/Passive/Resistor  R=0.005 kOhm  R_tol=5  enable_R_tol=0  tol_distribution=1  nSigma=4  enable_operating_limits=0  operating_limit_action=2  max_working_voltage=100 V  power_rating=1 W  enable_faults=0  fault_action=1  R_faulted=inf Ohm  enable_temporal_fault=0  t_fault=1 s  enable_behavioral_fault=0  max_permissible_current=1 A  t_fail_on_current=1 s  noise_mode=0  sample_time=1e-3 s  repeatability=1  auto_seed=2513690131  user_seed=0  Tdevice=25 degC  alpha=3.93e-3 1/K  Tmeas=25 degC  thermal_mass=100 J/K  power_derating_T1=70 degC  power_derating_T2=155 degC  operating_temperature_range_vec=[-50, 150] degC  temperature_specify=off  temperature_priority=High  temperature=298.15 K  temperature_nominal_specify=off  temperature_nominal_unit=K  temperature_nominal_value=1
  R-Visco LR1 : ee_lib/Passive/Resistor  Commented=on  R=0.005 kOhm  R_tol=5  enable_R_tol=0  tol_distribution=1  nSigma=4  enable_operating_limits=0  operating_limit_action=2  max_working_voltage=100 V  power_rating=1 W  enable_faults=0  fault_action=1  R_faulted=inf Ohm  enable_temporal_fault=0  t_fault=1 s  enable_behavioral_fault=0  max_permissible_current=1 A  t_fail_on_current=1 s  noise_mode=0  sample_time=1e-3 s  repeatability=1  auto_seed=894406345  user_seed=0  Tdevice=25 degC  alpha=3.93e-3 1/K  Tmeas=25 degC  thermal_mass=100 J/K  power_derating_T1=70 degC  power_derating_T2=155 degC  operating_temperature_range_vec=[-50, 150] degC  temperature_specify=off  temperature_priority=High  temperature=298.15 K  temperature_nominal_specify=off  temperature_nominal_unit=K  temperature_nominal_value=1
  R-Visco LR2 : ee_lib/Passive/Resistor  R=0.005 kOhm  R_tol=5  enable_R_tol=0  tol_distribution=1  nSigma=4  enable_operating_limits=0  operating_limit_action=2  max_working_voltage=100 V  power_rating=1 W  enable_faults=0  fault_action=1  R_faulted=inf Ohm  enable_temporal_fault=0  t_fault=1 s  enable_behavioral_fault=0  max_permissible_current=1 A  t_fail_on_current=1 s  noise_mode=0  sample_time=1e-3 s  repeatability=1  auto_seed=2361044919  user_seed=0  Tdevice=25 degC  alpha=3.93e-3 1/K  Tmeas=25 degC  thermal_mass=100 J/K  power_derating_T1=70 degC  power_derating_T2=155 degC  operating_temperature_range_vec=[-50, 150] degC  temperature_specify=off  temperature_priority=High  temperature=298.15 K  temperature_nominal_specify=off  temperature_nominal_unit=K  temperature_nominal_value=1
  R-Visco LR3 : ee_lib/Passive/Resistor  Commented=on  R=0.005 kOhm  R_tol=5  enable_R_tol=0  tol_distribution=1  nSigma=4  enable_operating_limits=0  operating_limit_action=2  max_working_voltage=100 V  power_rating=1 W  enable_faults=0  fault_action=1  R_faulted=inf Ohm  enable_temporal_fault=0  t_fault=1 s  enable_behavioral_fault=0  max_permissible_current=1 A  t_fail_on_current=1 s  noise_mode=0  sample_time=1e-3 s  repeatability=1  auto_seed=1717100866  user_seed=0  Tdevice=25 degC  alpha=3.93e-3 1/K  Tmeas=25 degC  thermal_mass=100 J/K  power_derating_T1=70 degC  power_derating_T2=155 degC  operating_temperature_range_vec=[-50, 150] degC  temperature_specify=off  temperature_priority=High  temperature=298.15 K  temperature_nominal_specify=off  temperature_nominal_unit=K  temperature_nominal_value=1
  R-Visco LR4 : ee_lib/Passive/Resistor  R=0.005 kOhm  R_tol=5  enable_R_tol=0  tol_distribution=1  nSigma=4  enable_operating_limits=0  operating_limit_action=2  max_working_voltage=100 V  power_rating=1 W  enable_faults=0  fault_action=1  R_faulted=inf Ohm  enable_temporal_fault=0  t_fault=1 s  enable_behavioral_fault=0  max_permissible_current=1 A  t_fail_on_current=1 s  noise_mode=0  sample_time=1e-3 s  repeatability=1  auto_seed=2361044919  user_seed=0  Tdevice=25 degC  alpha=3.93e-3 1/K  Tmeas=25 degC  thermal_mass=100 J/K  power_derating_T1=70 degC  power_derating_T2=155 degC  operating_temperature_range_vec=[-50, 150] degC  temperature_specify=off  temperature_priority=High  temperature=298.15 K  temperature_nominal_specify=off  temperature_nominal_unit=K  temperature_nominal_value=1
  R-Visco Left Gastric1 : ee_lib/Passive/Resistor  Commented=on  R=0.005 kOhm  R_tol=5  enable_R_tol=0  tol_distribution=1  nSigma=4  enable_operating_limits=0  operating_limit_action=2  max_working_voltage=100 V  power_rating=1 W  enable_faults=0  fault_action=1  R_faulted=inf Ohm  enable_temporal_fault=0  t_fault=1 s  enable_behavioral_fault=0  max_permissible_current=1 A  t_fail_on_current=1 s  noise_mode=0  sample_time=1e-3 s  repeatability=1  auto_seed=3252463469  user_seed=0  Tdevice=25 degC  alpha=3.93e-3 1/K  Tmeas=25 degC  thermal_mass=100 J/K  power_derating_T1=70 degC  power_derating_T2=155 degC  operating_temperature_range_vec=[-50, 150] degC  temperature_specify=off  temperature_priority=High  temperature=298.15 K  temperature_nominal_specify=off  temperature_nominal_unit=K  temperature_nominal_value=1
  R-Visco Left Gastric2 : ee_lib/Passive/Resistor  R=0.005 kOhm  R_tol=5  enable_R_tol=0  tol_distribution=1  nSigma=4  enable_operating_limits=0  operating_limit_action=2  max_working_voltage=100 V  power_rating=1 W  enable_faults=0  fault_action=1  R_faulted=inf Ohm  enable_temporal_fault=0  t_fault=1 s  enable_behavioral_fault=0  max_permissible_current=1 A  t_fail_on_current=1 s  noise_mode=0  sample_time=1e-3 s  repeatability=1  auto_seed=3939316790  user_seed=0  Tdevice=25 degC  alpha=3.93e-3 1/K  Tmeas=25 degC  thermal_mass=100 J/K  power_derating_T1=70 degC  power_derating_T2=155 degC  operating_temperature_range_vec=[-50, 150] degC  temperature_specify=off  temperature_priority=High  temperature=298.15 K  temperature_nominal_specify=off  temperature_nominal_unit=K  temperature_nominal_value=1
  R-Visco Left Gastric3 : ee_lib/Passive/Resistor  Commented=on  R=0.005 kOhm  R_tol=5  enable_R_tol=0  tol_distribution=1  nSigma=4  enable_operating_limits=0  operating_limit_action=2  max_working_voltage=100 V  power_rating=1 W  enable_faults=0  fault_action=1  R_faulted=inf Ohm  enable_temporal_fault=0  t_fault=1 s  enable_behavioral_fault=0  max_permissible_current=1 A  t_fail_on_current=1 s  noise_mode=0  sample_time=1e-3 s  repeatability=1  auto_seed=3243211774  user_seed=0  Tdevice=25 degC  alpha=3.93e-3 1/K  Tmeas=25 degC  thermal_mass=100 J/K  power_derating_T1=70 degC  power_derating_T2=155 degC  operating_temperature_range_vec=[-50, 150] degC  temperature_specify=off  temperature_priority=High  temperature=298.15 K  temperature_nominal_specify=off  temperature_nominal_unit=K  temperature_nominal_value=1
  R-Visco Left Gastric4 : ee_lib/Passive/Resistor  R=0.005 kOhm  R_tol=5  enable_R_tol=0  tol_distribution=1  nSigma=4  enable_operating_limits=0  operating_limit_action=2  max_working_voltage=100 V  power_rating=1 W  enable_faults=0  fault_action=1  R_faulted=inf Ohm  enable_temporal_fault=0  t_fault=1 s  enable_behavioral_fault=0  max_permissible_current=1 A  t_fail_on_current=1 s  noise_mode=0  sample_time=1e-3 s  repeatability=1  auto_seed=3939316790  user_seed=0  Tdevice=25 degC  alpha=3.93e-3 1/K  Tmeas=25 degC  thermal_mass=100 J/K  power_derating_T1=70 degC  power_derating_T2=155 degC  operating_temperature_range_vec=[-50, 150] degC  temperature_specify=off  temperature_priority=High  temperature=298.15 K  temperature_nominal_specify=off  temperature_nominal_unit=K  temperature_nominal_value=1
  R-Visco PT1 : ee_lib/Passive/Resistor  Commented=on  R=0.005 kOhm  R_tol=5  enable_R_tol=0  tol_distribution=1  nSigma=4  enable_operating_limits=0  operating_limit_action=2  max_working_voltage=100 V  power_rating=1 W  enable_faults=0  fault_action=1  R_faulted=inf Ohm  enable_temporal_fault=0  t_fault=1 s  enable_behavioral_fault=0  max_permissible_current=1 A  t_fail_on_current=1 s  noise_mode=0  sample_time=1e-3 s  repeatability=1  auto_seed=2348024382  user_seed=0  Tdevice=25 degC  alpha=3.93e-3 1/K  Tmeas=25 degC  thermal_mass=100 J/K  power_derating_T1=70 degC  power_derating_T2=155 degC  operating_temperature_range_vec=[-50, 150] degC  temperature_specify=off  temperature_priority=High  temperature=298.15 K  temperature_nominal_specify=off  temperature_nominal_unit=K  temperature_nominal_value=1
  R-Visco PT2 : ee_lib/Passive/Resistor  R=0.005 kOhm  R_tol=5  enable_R_tol=0  tol_distribution=1  nSigma=4  enable_operating_limits=0  operating_limit_action=2  max_working_voltage=100 V  power_rating=1 W  enable_faults=0  fault_action=1  R_faulted=inf Ohm  enable_temporal_fault=0  t_fault=1 s  enable_behavioral_fault=0  max_permissible_current=1 A  t_fail_on_current=1 s  noise_mode=0  sample_time=1e-3 s  repeatability=1  auto_seed=1227669238  user_seed=0  Tdevice=25 degC  alpha=3.93e-3 1/K  Tmeas=25 degC  thermal_mass=100 J/K  power_derating_T1=70 degC  power_derating_T2=155 degC  operating_temperature_range_vec=[-50, 150] degC  temperature_specify=off  temperature_priority=High  temperature=298.15 K  temperature_nominal_specify=off  temperature_nominal_unit=K  temperature_nominal_value=1
  R-Visco PT3 : ee_lib/Passive/Resistor  Commented=on  R=0.005 kOhm  R_tol=5  enable_R_tol=0  tol_distribution=1  nSigma=4  enable_operating_limits=0  operating_limit_action=2  max_working_voltage=100 V  power_rating=1 W  enable_faults=0  fault_action=1  R_faulted=inf Ohm  enable_temporal_fault=0  t_fault=1 s  enable_behavioral_fault=0  max_permissible_current=1 A  t_fail_on_current=1 s  noise_mode=0  sample_time=1e-3 s  repeatability=1  auto_seed=1267919064  user_seed=0  Tdevice=25 degC  alpha=3.93e-3 1/K  Tmeas=25 degC  thermal_mass=100 J/K  power_derating_T1=70 degC  power_derating_T2=155 degC  operating_temperature_range_vec=[-50, 150] degC  temperature_specify=off  temperature_priority=High  temperature=298.15 K  temperature_nominal_specify=off  temperature_nominal_unit=K  temperature_nominal_value=1
  R-Visco PT4 : ee_lib/Passive/Resistor  R=0.005 kOhm  R_tol=5  enable_R_tol=0  tol_distribution=1  nSigma=4  enable_operating_limits=0  operating_limit_action=2  max_working_voltage=100 V  power_rating=1 W  enable_faults=0  fault_action=1  R_faulted=inf Ohm  enable_temporal_fault=0  t_fault=1 s  enable_behavioral_fault=0  max_permissible_current=1 A  t_fail_on_current=1 s  noise_mode=0  sample_time=1e-3 s  repeatability=1  auto_seed=1227669238  user_seed=0  Tdevice=25 degC  alpha=3.93e-3 1/K  Tmeas=25 degC  thermal_mass=100 J/K  power_derating_T1=70 degC  power_derating_T2=155 degC  operating_temperature_range_vec=[-50, 150] degC  temperature_specify=off  temperature_priority=High  temperature=298.15 K  temperature_nominal_specify=off  temperature_nominal_unit=K  temperature_nominal_value=1
  R-Visco RCI1 : ee_lib/Passive/Resistor  Commented=on  R=0.005 kOhm  R_tol=5  enable_R_tol=0  tol_distribution=1  nSigma=4  enable_operating_limits=0  operating_limit_action=2  max_working_voltage=100 V  power_rating=1 W  enable_faults=0  fault_action=1  R_faulted=inf Ohm  enable_temporal_fault=0  t_fault=1 s  enable_behavioral_fault=0  max_permissible_current=1 A  t_fail_on_current=1 s  noise_mode=0  sample_time=1e-3 s  repeatability=1  auto_seed=1534970601  user_seed=0  Tdevice=25 degC  alpha=3.93e-3 1/K  Tmeas=25 degC  thermal_mass=100 J/K  power_derating_T1=70 degC  power_derating_T2=155 degC  operating_temperature_range_vec=[-50, 150] degC  temperature_specify=off  temperature_priority=High  temperature=298.15 K  temperature_nominal_specify=off  temperature_nominal_unit=K  temperature_nominal_value=1
  R-Visco RCI2 : ee_lib/Passive/Resistor  R=0.005 kOhm  R_tol=5  enable_R_tol=0  tol_distribution=1  nSigma=4  enable_operating_limits=0  operating_limit_action=2  max_working_voltage=100 V  power_rating=1 W  enable_faults=0  fault_action=1  R_faulted=inf Ohm  enable_temporal_fault=0  t_fault=1 s  enable_behavioral_fault=0  max_permissible_current=1 A  t_fail_on_current=1 s  noise_mode=0  sample_time=1e-3 s  repeatability=1  auto_seed=3252150220  user_seed=0  Tdevice=25 degC  alpha=3.93e-3 1/K  Tmeas=25 degC  thermal_mass=100 J/K  power_derating_T1=70 degC  power_derating_T2=155 degC  operating_temperature_range_vec=[-50, 150] degC  temperature_specify=off  temperature_priority=High  temperature=298.15 K  temperature_nominal_specify=off  temperature_nominal_unit=K  temperature_nominal_value=1
  R-Visco RCI3 : ee_lib/Passive/Resistor  Commented=on  R=0.005 kOhm  R_tol=5  enable_R_tol=0  tol_distribution=1  nSigma=4  enable_operating_limits=0  operating_limit_action=2  max_working_voltage=100 V  power_rating=1 W  enable_faults=0  fault_action=1  R_faulted=inf Ohm  enable_temporal_fault=0  t_fault=1 s  enable_behavioral_fault=0  max_permissible_current=1 A  t_fail_on_current=1 s  noise_mode=0  sample_time=1e-3 s  repeatability=1  auto_seed=2748804455  user_seed=0  Tdevice=25 degC  alpha=3.93e-3 1/K  Tmeas=25 degC  thermal_mass=100 J/K  power_derating_T1=70 degC  power_derating_T2=155 degC  operating_temperature_range_vec=[-50, 150] degC  temperature_specify=off  temperature_priority=High  temperature=298.15 K  temperature_nominal_specify=off  temperature_nominal_unit=K  temperature_nominal_value=1
  R-Visco RCI4 : ee_lib/Passive/Resistor  R=0.005 kOhm  R_tol=5  enable_R_tol=0  tol_distribution=1  nSigma=4  enable_operating_limits=0  operating_limit_action=2  max_working_voltage=100 V  power_rating=1 W  enable_faults=0  fault_action=1  R_faulted=inf Ohm  enable_temporal_fault=0  t_fault=1 s  enable_behavioral_fault=0  max_permissible_current=1 A  t_fail_on_current=1 s  noise_mode=0  sample_time=1e-3 s  repeatability=1  auto_seed=3252150220  user_seed=0  Tdevice=25 degC  alpha=3.93e-3 1/K  Tmeas=25 degC  thermal_mass=100 J/K  power_derating_T1=70 degC  power_derating_T2=155 degC  operating_temperature_range_vec=[-50, 150] degC  temperature_specify=off  temperature_priority=High  temperature=298.15 K  temperature_nominal_specify=off  temperature_nominal_unit=K  temperature_nominal_value=1
  R-Visco REI1 : ee_lib/Passive/Resistor  Commented=on  R=0.005 kOhm  R_tol=5  enable_R_tol=0  tol_distribution=1  nSigma=4  enable_operating_limits=0  operating_limit_action=2  max_working_voltage=100 V  power_rating=1 W  enable_faults=0  fault_action=1  R_faulted=inf Ohm  enable_temporal_fault=0  t_fault=1 s  enable_behavioral_fault=0  max_permissible_current=1 A  t_fail_on_current=1 s  noise_mode=0  sample_time=1e-3 s  repeatability=1  auto_seed=3010762581  user_seed=0  Tdevice=25 degC  alpha=3.93e-3 1/K  Tmeas=25 degC  thermal_mass=100 J/K  power_derating_T1=70 degC  power_derating_T2=155 degC  operating_temperature_range_vec=[-50, 150] degC  temperature_specify=off  temperature_priority=High  temperature=298.15 K  temperature_nominal_specify=off  temperature_nominal_unit=K  temperature_nominal_value=1
  R-Visco REI2 : ee_lib/Passive/Resistor  R=0.005 kOhm  R_tol=5  enable_R_tol=0  tol_distribution=1  nSigma=4  enable_operating_limits=0  operating_limit_action=2  max_working_voltage=100 V  power_rating=1 W  enable_faults=0  fault_action=1  R_faulted=inf Ohm  enable_temporal_fault=0  t_fault=1 s  enable_behavioral_fault=0  max_permissible_current=1 A  t_fail_on_current=1 s  noise_mode=0  sample_time=1e-3 s  repeatability=1  auto_seed=3237241810  user_seed=0  Tdevice=25 degC  alpha=3.93e-3 1/K  Tmeas=25 degC  thermal_mass=100 J/K  power_derating_T1=70 degC  power_derating_T2=155 degC  operating_temperature_range_vec=[-50, 150] degC  temperature_specify=off  temperature_priority=High  temperature=298.15 K  temperature_nominal_specify=off  temperature_nominal_unit=K  temperature_nominal_value=1
  R-Visco REI3 : ee_lib/Passive/Resistor  Commented=on  R=0.005 kOhm  R_tol=5  enable_R_tol=0  tol_distribution=1  nSigma=4  enable_operating_limits=0  operating_limit_action=2  max_working_voltage=100 V  power_rating=1 W  enable_faults=0  fault_action=1  R_faulted=inf Ohm  enable_temporal_fault=0  t_fault=1 s  enable_behavioral_fault=0  max_permissible_current=1 A  t_fail_on_current=1 s  noise_mode=0  sample_time=1e-3 s  repeatability=1  auto_seed=3801549231  user_seed=0  Tdevice=25 degC  alpha=3.93e-3 1/K  Tmeas=25 degC  thermal_mass=100 J/K  power_derating_T1=70 degC  power_derating_T2=155 degC  operating_temperature_range_vec=[-50, 150] degC  temperature_specify=off  temperature_priority=High  temperature=298.15 K  temperature_nominal_specify=off  temperature_nominal_unit=K  temperature_nominal_value=1
  R-Visco REI4 : ee_lib/Passive/Resistor  R=0.005 kOhm  R_tol=5  enable_R_tol=0  tol_distribution=1  nSigma=4  enable_operating_limits=0  operating_limit_action=2  max_working_voltage=100 V  power_rating=1 W  enable_faults=0  fault_action=1  R_faulted=inf Ohm  enable_temporal_fault=0  t_fault=1 s  enable_behavioral_fault=0  max_permissible_current=1 A  t_fail_on_current=1 s  noise_mode=0  sample_time=1e-3 s  repeatability=1  auto_seed=3237241810  user_seed=0  Tdevice=25 degC  alpha=3.93e-3 1/K  Tmeas=25 degC  thermal_mass=100 J/K  power_derating_T1=70 degC  power_derating_T2=155 degC  operating_temperature_range_vec=[-50, 150] degC  temperature_specify=off  temperature_priority=High  temperature=298.15 K  temperature_nominal_specify=off  temperature_nominal_unit=K  temperature_nominal_value=1
  R-Visco RFA1 : ee_lib/Passive/Resistor  Commented=on  R=0.005 kOhm  R_tol=5  enable_R_tol=0  tol_distribution=1  nSigma=4  enable_operating_limits=0  operating_limit_action=2  max_working_voltage=100 V  power_rating=1 W  enable_faults=0  fault_action=1  R_faulted=inf Ohm  enable_temporal_fault=0  t_fault=1 s  enable_behavioral_fault=0  max_permissible_current=1 A  t_fail_on_current=1 s  noise_mode=0  sample_time=1e-3 s  repeatability=1  auto_seed=469107052  user_seed=0  Tdevice=25 degC  alpha=3.93e-3 1/K  Tmeas=25 degC  thermal_mass=100 J/K  power_derating_T1=70 degC  power_derating_T2=155 degC  operating_temperature_range_vec=[-50, 150] degC  temperature_specify=off  temperature_priority=High  temperature=298.15 K  temperature_nominal_specify=off  temperature_nominal_unit=K  temperature_nominal_value=1
  R-Visco RFA2 : ee_lib/Passive/Resistor  R=0.005 kOhm  R_tol=5  enable_R_tol=0  tol_distribution=1  nSigma=4  enable_operating_limits=0  operating_limit_action=2  max_working_voltage=100 V  power_rating=1 W  enable_faults=0  fault_action=1  R_faulted=inf Ohm  enable_temporal_fault=0  t_fault=1 s  enable_behavioral_fault=0  max_permissible_current=1 A  t_fail_on_current=1 s  noise_mode=0  sample_time=1e-3 s  repeatability=1  auto_seed=1634002471  user_seed=0  Tdevice=25 degC  alpha=3.93e-3 1/K  Tmeas=25 degC  thermal_mass=100 J/K  power_derating_T1=70 degC  power_derating_T2=155 degC  operating_temperature_range_vec=[-50, 150] degC  temperature_specify=off  temperature_priority=High  temperature=298.15 K  temperature_nominal_specify=off  temperature_nominal_unit=K  temperature_nominal_value=1
  R-Visco RFA3 : ee_lib/Passive/Resistor  Commented=on  R=0.005 kOhm  R_tol=5  enable_R_tol=0  tol_distribution=1  nSigma=4  enable_operating_limits=0  operating_limit_action=2  max_working_voltage=100 V  power_rating=1 W  enable_faults=0  fault_action=1  R_faulted=inf Ohm  enable_temporal_fault=0  t_fault=1 s  enable_behavioral_fault=0  max_permissible_current=1 A  t_fail_on_current=1 s  noise_mode=0  sample_time=1e-3 s  repeatability=1  auto_seed=900411215  user_seed=0  Tdevice=25 degC  alpha=3.93e-3 1/K  Tmeas=25 degC  thermal_mass=100 J/K  power_derating_T1=70 degC  power_derating_T2=155 degC  operating_temperature_range_vec=[-50, 150] degC  temperature_specify=off  temperature_priority=High  temperature=298.15 K  temperature_nominal_specify=off  temperature_nominal_unit=K  temperature_nominal_value=1
  R-Visco RFA4 : ee_lib/Passive/Resistor  R=0.005 kOhm  R_tol=5  enable_R_tol=0  tol_distribution=1  nSigma=4  enable_operating_limits=0  operating_limit_action=2  max_working_voltage=100 V  power_rating=1 W  enable_faults=0  fault_action=1  R_faulted=inf Ohm  enable_temporal_fault=0  t_fault=1 s  enable_behavioral_fault=0  max_permissible_current=1 A  t_fail_on_current=1 s  noise_mode=0  sample_time=1e-3 s  repeatability=1  auto_seed=1634002471  user_seed=0  Tdevice=25 degC  alpha=3.93e-3 1/K  Tmeas=25 degC  thermal_mass=100 J/K  power_derating_T1=70 degC  power_derating_T2=155 degC  operating_temperature_range_vec=[-50, 150] degC  temperature_specify=off  temperature_priority=High  temperature=298.15 K  temperature_nominal_specify=off  temperature_nominal_unit=K  temperature_nominal_value=1
  R-Visco RR1 : ee_lib/Passive/Resistor  Commented=on  R=0.005 kOhm  R_tol=5  enable_R_tol=0  tol_distribution=1  nSigma=4  enable_operating_limits=0  operating_limit_action=2  max_working_voltage=100 V  power_rating=1 W  enable_faults=0  fault_action=1  R_faulted=inf Ohm  enable_temporal_fault=0  t_fault=1 s  enable_behavioral_fault=0  max_permissible_current=1 A  t_fail_on_current=1 s  noise_mode=0  sample_time=1e-3 s  repeatability=1  auto_seed=28393024  user_seed=0  Tdevice=25 degC  alpha=3.93e-3 1/K  Tmeas=25 degC  thermal_mass=100 J/K  power_derating_T1=70 degC  power_derating_T2=155 degC  operating_temperature_range_vec=[-50, 150] degC  temperature_specify=off  temperature_priority=High  temperature=298.15 K  temperature_nominal_specify=off  temperature_nominal_unit=K  temperature_nominal_value=1
  R-Visco RR2 : ee_lib/Passive/Resistor  R=0.005 kOhm  R_tol=5  enable_R_tol=0  tol_distribution=1  nSigma=4  enable_operating_limits=0  operating_limit_action=2  max_working_voltage=100 V  power_rating=1 W  enable_faults=0  fault_action=1  R_faulted=inf Ohm  enable_temporal_fault=0  t_fault=1 s  enable_behavioral_fault=0  max_permissible_current=1 A  t_fail_on_current=1 s  noise_mode=0  sample_time=1e-3 s  repeatability=1  auto_seed=2438775377  user_seed=0  Tdevice=25 degC  alpha=3.93e-3 1/K  Tmeas=25 degC  thermal_mass=100 J/K  power_derating_T1=70 degC  power_derating_T2=155 degC  operating_temperature_range_vec=[-50, 150] degC  temperature_specify=off  temperature_priority=High  temperature=298.15 K  temperature_nominal_specify=off  temperature_nominal_unit=K  temperature_nominal_value=1
  R-Visco RR3 : ee_lib/Passive/Resistor  Commented=on  R=0.005 kOhm  R_tol=5  enable_R_tol=0  tol_distribution=1  nSigma=4  enable_operating_limits=0  operating_limit_action=2  max_working_voltage=100 V  power_rating=1 W  enable_faults=0  fault_action=1  R_faulted=inf Ohm  enable_temporal_fault=0  t_fault=1 s  enable_behavioral_fault=0  max_permissible_current=1 A  t_fail_on_current=1 s  noise_mode=0  sample_time=1e-3 s  repeatability=1  auto_seed=2063115406  user_seed=0  Tdevice=25 degC  alpha=3.93e-3 1/K  Tmeas=25 degC  thermal_mass=100 J/K  power_derating_T1=70 degC  power_derating_T2=155 degC  operating_temperature_range_vec=[-50, 150] degC  temperature_specify=off  temperature_priority=High  temperature=298.15 K  temperature_nominal_specify=off  temperature_nominal_unit=K  temperature_nominal_value=1
  R-Visco RR4 : ee_lib/Passive/Resistor  R=0.005 kOhm  R_tol=5  enable_R_tol=0  tol_distribution=1  nSigma=4  enable_operating_limits=0  operating_limit_action=2  max_working_voltage=100 V  power_rating=1 W  enable_faults=0  fault_action=1  R_faulted=inf Ohm  enable_temporal_fault=0  t_fault=1 s  enable_behavioral_fault=0  max_permissible_current=1 A  t_fail_on_current=1 s  noise_mode=0  sample_time=1e-3 s  repeatability=1  auto_seed=2438775377  user_seed=0  Tdevice=25 degC  alpha=3.93e-3 1/K  Tmeas=25 degC  thermal_mass=100 J/K  power_derating_T1=70 degC  power_derating_T2=155 degC  operating_temperature_range_vec=[-50, 150] degC  temperature_specify=off  temperature_priority=High  temperature=298.15 K  temperature_nominal_specify=off  temperature_nominal_unit=K  temperature_nominal_value=1
  R-Visco Right Gastric1 : ee_lib/Passive/Resistor  Commented=on  R=.005 kOhm  R_tol=5  enable_R_tol=0  tol_distribution=1  nSigma=4  enable_operating_limits=0  operating_limit_action=2  max_working_voltage=100 V  power_rating=1 W  enable_faults=0  fault_action=1  R_faulted=inf Ohm  enable_temporal_fault=0  t_fault=1 s  enable_behavioral_fault=0  max_permissible_current=1 A  t_fail_on_current=1 s  noise_mode=0  sample_time=1e-3 s  repeatability=1  auto_seed=2565392898  user_seed=0  Tdevice=25 degC  alpha=3.93e-3 1/K  Tmeas=25 degC  thermal_mass=100 J/K  power_derating_T1=70 degC  power_derating_T2=155 degC  operating_temperature_range_vec=[-50, 150] degC  temperature_specify=off  temperature_priority=High  temperature=298.15 K  temperature_nominal_specify=off  temperature_nominal_unit=K  temperature_nominal_value=1
  R-Visco Right Gastric2 : ee_lib/Passive/Resistor  R=.005 kOhm  R_tol=5  enable_R_tol=0  tol_distribution=1  nSigma=4  enable_operating_limits=0  operating_limit_action=2  max_working_voltage=100 V  power_rating=1 W  enable_faults=0  fault_action=1  R_faulted=inf Ohm  enable_temporal_fault=0  t_fault=1 s  enable_behavioral_fault=0  max_permissible_current=1 A  t_fail_on_current=1 s  noise_mode=0  sample_time=1e-3 s  repeatability=1  auto_seed=325791693  user_seed=0  Tdevice=25 degC  alpha=3.93e-3 1/K  Tmeas=25 degC  thermal_mass=100 J/K  power_derating_T1=70 degC  power_derating_T2=155 degC  operating_temperature_range_vec=[-50, 150] degC  temperature_specify=off  temperature_priority=High  temperature=298.15 K  temperature_nominal_specify=off  temperature_nominal_unit=K  temperature_nominal_value=1
  R-Visco Right Gastric3 : ee_lib/Passive/Resistor  Commented=on  R=.005 kOhm  R_tol=5  enable_R_tol=0  tol_distribution=1  nSigma=4  enable_operating_limits=0  operating_limit_action=2  max_working_voltage=100 V  power_rating=1 W  enable_faults=0  fault_action=1  R_faulted=inf Ohm  enable_temporal_fault=0  t_fault=1 s  enable_behavioral_fault=0  max_permissible_current=1 A  t_fail_on_current=1 s  noise_mode=0  sample_time=1e-3 s  repeatability=1  auto_seed=485277873  user_seed=0  Tdevice=25 degC  alpha=3.93e-3 1/K  Tmeas=25 degC  thermal_mass=100 J/K  power_derating_T1=70 degC  power_derating_T2=155 degC  operating_temperature_range_vec=[-50, 150] degC  temperature_specify=off  temperature_priority=High  temperature=298.15 K  temperature_nominal_specify=off  temperature_nominal_unit=K  temperature_nominal_value=1
  R-Visco Right Gastric4 : ee_lib/Passive/Resistor  R=.005 kOhm  R_tol=5  enable_R_tol=0  tol_distribution=1  nSigma=4  enable_operating_limits=0  operating_limit_action=2  max_working_voltage=100 V  power_rating=1 W  enable_faults=0  fault_action=1  R_faulted=inf Ohm  enable_temporal_fault=0  t_fault=1 s  enable_behavioral_fault=0  max_permissible_current=1 A  t_fail_on_current=1 s  noise_mode=0  sample_time=1e-3 s  repeatability=1  auto_seed=325791693  user_seed=0  Tdevice=25 degC  alpha=3.93e-3 1/K  Tmeas=25 degC  thermal_mass=100 J/K  power_derating_T1=70 degC  power_derating_T2=155 degC  operating_temperature_range_vec=[-50, 150] degC  temperature_specify=off  temperature_priority=High  temperature=298.15 K  temperature_nominal_specify=off  temperature_nominal_unit=K  temperature_nominal_value=1
  R-Visco SM1 : ee_lib/Passive/Resistor  Commented=on  R=0.005 kOhm  R_tol=5  enable_R_tol=0  tol_distribution=1  nSigma=4  enable_operating_limits=0  operating_limit_action=2  max_working_voltage=100 V  power_rating=1 W  enable_faults=0  fault_action=1  R_faulted=inf Ohm  enable_temporal_fault=0  t_fault=1 s  enable_behavioral_fault=0  max_permissible_current=1 A  t_fail_on_current=1 s  noise_mode=0  sample_time=1e-3 s  repeatability=1  auto_seed=2831139648  user_seed=0  Tdevice=25 degC  alpha=3.93e-3 1/K  Tmeas=25 degC  thermal_mass=100 J/K  power_derating_T1=70 degC  power_derating_T2=155 degC  operating_temperature_range_vec=[-50, 150] degC  temperature_specify=off  temperature_priority=High  temperature=298.15 K  temperature_nominal_specify=off  temperature_nominal_unit=K  temperature_nominal_value=1
  R-Visco SM2 : ee_lib/Passive/Resistor  R=0.005 kOhm  R_tol=5  enable_R_tol=0  tol_distribution=1  nSigma=4  enable_operating_limits=0  operating_limit_action=2  max_working_voltage=100 V  power_rating=1 W  enable_faults=0  fault_action=1  R_faulted=inf Ohm  enable_temporal_fault=0  t_fault=1 s  enable_behavioral_fault=0  max_permissible_current=1 A  t_fail_on_current=1 s  noise_mode=0  sample_time=1e-3 s  repeatability=1  auto_seed=231713996  user_seed=0  Tdevice=25 degC  alpha=3.93e-3 1/K  Tmeas=25 degC  thermal_mass=100 J/K  power_derating_T1=70 degC  power_derating_T2=155 degC  operating_temperature_range_vec=[-50, 150] degC  temperature_specify=off  temperature_priority=High  temperature=298.15 K  temperature_nominal_specify=off  temperature_nominal_unit=K  temperature_nominal_value=1
  R-Visco SM3 : ee_lib/Passive/Resistor  Commented=on  R=0.005 kOhm  R_tol=5  enable_R_tol=0  tol_distribution=1  nSigma=4  enable_operating_limits=0  operating_limit_action=2  max_working_voltage=100 V  power_rating=1 W  enable_faults=0  fault_action=1  R_faulted=inf Ohm  enable_temporal_fault=0  t_fault=1 s  enable_behavioral_fault=0  max_permissible_current=1 A  t_fail_on_current=1 s  noise_mode=0  sample_time=1e-3 s  repeatability=1  auto_seed=568523275  user_seed=0  Tdevice=25 degC  alpha=3.93e-3 1/K  Tmeas=25 degC  thermal_mass=100 J/K  power_derating_T1=70 degC  power_derating_T2=155 degC  operating_temperature_range_vec=[-50, 150] degC  temperature_specify=off  temperature_priority=High  temperature=298.15 K  temperature_nominal_specify=off  temperature_nominal_unit=K  temperature_nominal_value=1
  R-Visco SM4 : ee_lib/Passive/Resistor  R=0.005 kOhm  R_tol=5  enable_R_tol=0  tol_distribution=1  nSigma=4  enable_operating_limits=0  operating_limit_action=2  max_working_voltage=100 V  power_rating=1 W  enable_faults=0  fault_action=1  R_faulted=inf Ohm  enable_temporal_fault=0  t_fault=1 s  enable_behavioral_fault=0  max_permissible_current=1 A  t_fail_on_current=1 s  noise_mode=0  sample_time=1e-3 s  repeatability=1  auto_seed=231713996  user_seed=0  Tdevice=25 degC  alpha=3.93e-3 1/K  Tmeas=25 degC  thermal_mass=100 J/K  power_derating_T1=70 degC  power_derating_T2=155 degC  operating_temperature_range_vec=[-50, 150] degC  temperature_specify=off  temperature_priority=High  temperature=298.15 K  temperature_nominal_specify=off  temperature_nominal_unit=K  temperature_nominal_value=1
  R-Visco Splentic1 : ee_lib/Passive/Resistor  Commented=on  R=0.005 kOhm  R_tol=5  enable_R_tol=0  tol_distribution=1  nSigma=4  enable_operating_limits=0  operating_limit_action=2  max_working_voltage=100 V  power_rating=1 W  enable_faults=0  fault_action=1  R_faulted=inf Ohm  enable_temporal_fault=0  t_fault=1 s  enable_behavioral_fault=0  max_permissible_current=1 A  t_fail_on_current=1 s  noise_mode=0  sample_time=1e-3 s  repeatability=1  auto_seed=2491108651  user_seed=0  Tdevice=25 degC  alpha=3.93e-3 1/K  Tmeas=25 degC  thermal_mass=100 J/K  power_derating_T1=70 degC  power_derating_T2=155 degC  operating_temperature_range_vec=[-50, 150] degC  temperature_specify=off  temperature_priority=High  temperature=298.15 K  temperature_nominal_specify=off  temperature_nominal_unit=K  temperature_nominal_value=1
  R-Visco Splentic2 : ee_lib/Passive/Resistor  R=0.005 kOhm  R_tol=5  enable_R_tol=0  tol_distribution=1  nSigma=4  enable_operating_limits=0  operating_limit_action=2  max_working_voltage=100 V  power_rating=1 W  enable_faults=0  fault_action=1  R_faulted=inf Ohm  enable_temporal_fault=0  t_fault=1 s  enable_behavioral_fault=0  max_permissible_current=1 A  t_fail_on_current=1 s  noise_mode=0  sample_time=1e-3 s  repeatability=1  auto_seed=2279758131  user_seed=0  Tdevice=25 degC  alpha=3.93e-3 1/K  Tmeas=25 degC  thermal_mass=100 J/K  power_derating_T1=70 degC  power_derating_T2=155 degC  operating_temperature_range_vec=[-50, 150] degC  temperature_specify=off  temperature_priority=High  temperature=298.15 K  temperature_nominal_specify=off  temperature_nominal_unit=K  temperature_nominal_value=1
  R-Visco Splentic3 : ee_lib/Passive/Resistor  Commented=on  R=0.005 kOhm  R_tol=5  enable_R_tol=0  tol_distribution=1  nSigma=4  enable_operating_limits=0  operating_limit_action=2  max_working_voltage=100 V  power_rating=1 W  enable_faults=0  fault_action=1  R_faulted=inf Ohm  enable_temporal_fault=0  t_fault=1 s  enable_behavioral_fault=0  max_permissible_current=1 A  t_fail_on_current=1 s  noise_mode=0  sample_time=1e-3 s  repeatability=1  auto_seed=274887603  user_seed=0  Tdevice=25 degC  alpha=3.93e-3 1/K  Tmeas=25 degC  thermal_mass=100 J/K  power_derating_T1=70 degC  power_derating_T2=155 degC  operating_temperature_range_vec=[-50, 150] degC  temperature_specify=off  temperature_priority=High  temperature=298.15 K  temperature_nominal_specify=off  temperature_nominal_unit=K  temperature_nominal_value=1
  R-Visco Splentic4 : ee_lib/Passive/Resistor  R=0.005 kOhm  R_tol=5  enable_R_tol=0  tol_distribution=1  nSigma=4  enable_operating_limits=0  operating_limit_action=2  max_working_voltage=100 V  power_rating=1 W  enable_faults=0  fault_action=1  R_faulted=inf Ohm  enable_temporal_fault=0  t_fault=1 s  enable_behavioral_fault=0  max_permissible_current=1 A  t_fail_on_current=1 s  noise_mode=0  sample_time=1e-3 s  repeatability=1  auto_seed=2279758131  user_seed=0  Tdevice=25 degC  alpha=3.93e-3 1/K  Tmeas=25 degC  thermal_mass=100 J/K  power_derating_T1=70 degC  power_derating_T2=155 degC  operating_temperature_range_vec=[-50, 150] degC  temperature_specify=off  temperature_priority=High  temperature=298.15 K  temperature_nominal_specify=off  temperature_nominal_unit=K  temperature_nominal_value=1
  R-Viscoelastic AB2 : ee_lib/Passive/Resistor  Commented=on  R=0.005 kOhm  R_tol=5  enable_R_tol=0  tol_distribution=1  nSigma=4  enable_operating_limits=0  operating_limit_action=2  max_working_voltage=100 V  power_rating=1 W  enable_faults=0  fault_action=1  R_faulted=inf Ohm  enable_temporal_fault=0  t_fault=1 s  enable_behavioral_fault=0  max_permissible_current=1 A  t_fail_on_current=1 s  noise_mode=0  sample_time=1e-3 s  repeatability=1  auto_seed=3908212406  user_seed=0  Tdevice=25 degC  alpha=3.93e-3 1/K  Tmeas=25 degC  thermal_mass=100 J/K  power_derating_T1=70 degC  power_derating_T2=155 degC  operating_temperature_range_vec=[-50, 150] degC  temperature_specify=off  temperature_priority=High  temperature=298.15 K  temperature_nominal_specify=off  temperature_nominal_unit=K  temperature_nominal_value=1
  R-Viscoelastic AB3 : ee_lib/Passive/Resistor  R=0.005 kOhm  R_tol=5  enable_R_tol=0  tol_distribution=1  nSigma=4  enable_operating_limits=0  operating_limit_action=2  max_working_voltage=100 V  power_rating=1 W  enable_faults=0  fault_action=1  R_faulted=inf Ohm  enable_temporal_fault=0  t_fault=1 s  enable_behavioral_fault=0  max_permissible_current=1 A  t_fail_on_current=1 s  noise_mode=0  sample_time=1e-3 s  repeatability=1  auto_seed=3346497771  user_seed=0  Tdevice=25 degC  alpha=3.93e-3 1/K  Tmeas=25 degC  thermal_mass=100 J/K  power_derating_T1=70 degC  power_derating_T2=155 degC  operating_temperature_range_vec=[-50, 150] degC  temperature_specify=off  temperature_priority=High  temperature=298.15 K  temperature_nominal_specify=off  temperature_nominal_unit=K  temperature_nominal_value=1
  R-Viscoelastic AB4 : ee_lib/Passive/Resistor  Commented=on  R=0.005 kOhm  R_tol=5  enable_R_tol=0  tol_distribution=1  nSigma=4  enable_operating_limits=0  operating_limit_action=2  max_working_voltage=100 V  power_rating=1 W  enable_faults=0  fault_action=1  R_faulted=inf Ohm  enable_temporal_fault=0  t_fault=1 s  enable_behavioral_fault=0  max_permissible_current=1 A  t_fail_on_current=1 s  noise_mode=0  sample_time=1e-3 s  repeatability=1  auto_seed=340579721  user_seed=0  Tdevice=25 degC  alpha=3.93e-3 1/K  Tmeas=25 degC  thermal_mass=100 J/K  power_derating_T1=70 degC  power_derating_T2=155 degC  operating_temperature_range_vec=[-50, 150] degC  temperature_specify=off  temperature_priority=High  temperature=298.15 K  temperature_nominal_specify=off  temperature_nominal_unit=K  temperature_nominal_value=1
  R-Viscoelastic AB5 : ee_lib/Passive/Resistor  R=0.005 kOhm  R_tol=5  enable_R_tol=0  tol_distribution=1  nSigma=4  enable_operating_limits=0  operating_limit_action=2  max_working_voltage=100 V  power_rating=1 W  enable_faults=0  fault_action=1  R_faulted=inf Ohm  enable_temporal_fault=0  t_fault=1 s  enable_behavioral_fault=0  max_permissible_current=1 A  t_fail_on_current=1 s  noise_mode=0  sample_time=1e-3 s  repeatability=1  auto_seed=3346497771  user_seed=0  Tdevice=25 degC  alpha=3.93e-3 1/K  Tmeas=25 degC  thermal_mass=100 J/K  power_derating_T1=70 degC  power_derating_T2=155 degC  operating_temperature_range_vec=[-50, 150] degC  temperature_specify=off  temperature_priority=High  temperature=298.15 K  temperature_nominal_specify=off  temperature_nominal_unit=K  temperature_nominal_value=1
  R-Viscoelastic DA1 : ee_lib/Passive/Resistor  Commented=on  R=0.005 kOhm  R_tol=5  enable_R_tol=0  tol_distribution=1  nSigma=4  enable_operating_limits=0  operating_limit_action=2  max_working_voltage=100 V  power_rating=1 W  enable_faults=0  fault_action=1  R_faulted=inf Ohm  enable_temporal_fault=0  t_fault=1 s  enable_behavioral_fault=0  max_permissible_current=1 A  t_fail_on_current=1 s  noise_mode=0  sample_time=1e-3 s  repeatability=1  auto_seed=2731625623  user_seed=0  Tdevice=25 degC  alpha=3.93e-3 1/K  Tmeas=25 degC  thermal_mass=100 J/K  power_derating_T1=70 degC  power_derating_T2=155 degC  operating_temperature_range_vec=[-50, 150] degC  temperature_specify=off  temperature_priority=High  temperature=298.15 K  temperature_nominal_specify=off  temperature_nominal_unit=K  temperature_nominal_value=1
  R-Viscoelastic DA2 : ee_lib/Passive/Resistor  R=0.005 kOhm  R_tol=5  enable_R_tol=0  tol_distribution=1  nSigma=4  enable_operating_limits=0  operating_limit_action=2  max_working_voltage=100 V  power_rating=1 W  enable_faults=0  fault_action=1  R_faulted=inf Ohm  enable_temporal_fault=0  t_fault=1 s  enable_behavioral_fault=0  max_permissible_current=1 A  t_fail_on_current=1 s  noise_mode=0  sample_time=1e-3 s  repeatability=1  auto_seed=4011545342  user_seed=0  Tdevice=25 degC  alpha=3.93e-3 1/K  Tmeas=25 degC  thermal_mass=100 J/K  power_derating_T1=70 degC  power_derating_T2=155 degC  operating_temperature_range_vec=[-50, 150] degC  temperature_specify=off  temperature_priority=High  temperature=298.15 K  temperature_nominal_specify=off  temperature_nominal_unit=K  temperature_nominal_value=1
  R-Viscoelastic DA3 : ee_lib/Passive/Resistor  Commented=on  R=0.005 kOhm  R_tol=5  enable_R_tol=0  tol_distribution=1  nSigma=4  enable_operating_limits=0  operating_limit_action=2  max_working_voltage=100 V  power_rating=1 W  enable_faults=0  fault_action=1  R_faulted=inf Ohm  enable_temporal_fault=0  t_fault=1 s  enable_behavioral_fault=0  max_permissible_current=1 A  t_fail_on_current=1 s  noise_mode=0  sample_time=1e-3 s  repeatability=1  auto_seed=2692747630  user_seed=0  Tdevice=25 degC  alpha=3.93e-3 1/K  Tmeas=25 degC  thermal_mass=100 J/K  power_derating_T1=70 degC  power_derating_T2=155 degC  operating_temperature_range_vec=[-50, 150] degC  temperature_specify=off  temperature_priority=High  temperature=298.15 K  temperature_nominal_specify=off  temperature_nominal_unit=K  temperature_nominal_value=1
  R-Viscoelastic DA4 : ee_lib/Passive/Resistor  R=0.005 kOhm  R_tol=5  enable_R_tol=0  tol_distribution=1  nSigma=4  enable_operating_limits=0  operating_limit_action=2  max_working_voltage=100 V  power_rating=1 W  enable_faults=0  fault_action=1  R_faulted=inf Ohm  enable_temporal_fault=0  t_fault=1 s  enable_behavioral_fault=0  max_permissible_current=1 A  t_fail_on_current=1 s  noise_mode=0  sample_time=1e-3 s  repeatability=1  auto_seed=4011545342  user_seed=0  Tdevice=25 degC  alpha=3.93e-3 1/K  Tmeas=25 degC  thermal_mass=100 J/K  power_derating_T1=70 degC  power_derating_T2=155 degC  operating_temperature_range_vec=[-50, 150] degC  temperature_specify=off  temperature_priority=High  temperature=298.15 K  temperature_nominal_specify=off  temperature_nominal_unit=K  temperature_nominal_value=1
  Resistor10 : ee_lib/Passive/Resistor  R=0.5 kOhm  R_tol=5  enable_R_tol=0  tol_distribution=1  nSigma=4  enable_operating_limits=0  operating_limit_action=2  max_working_voltage=100 V  power_rating=1 W  enable_faults=0  fault_action=1  R_faulted=inf Ohm  enable_temporal_fault=0  t_fault=1 s  enable_behavioral_fault=0  max_permissible_current=1 A  t_fail_on_current=1 s  noise_mode=0  sample_time=1e-3 s  repeatability=1  auto_seed=557942917  user_seed=0  Tdevice=25 degC  alpha=3.93e-3 1/K  Tmeas=25 degC  thermal_mass=100 J/K  power_derating_T1=70 degC  power_derating_T2=155 degC  operating_temperature_range_vec=[-50, 150] degC  temperature_specify=off  temperature_priority=High  temperature=298.15 K  temperature_nominal_specify=off  temperature_nominal_unit=K  temperature_nominal_value=1
  Resistor11 : ee_lib/Passive/Resistor  R=0.01 kOhm  R_tol=5  enable_R_tol=0  tol_distribution=1  nSigma=4  enable_operating_limits=0  operating_limit_action=2  max_working_voltage=100 V  power_rating=1 W  enable_faults=0  fault_action=1  R_faulted=inf Ohm  enable_temporal_fault=0  t_fault=1 s  enable_behavioral_fault=0  max_permissible_current=1 A  t_fail_on_current=1 s  noise_mode=0  sample_time=1e-3 s  repeatability=1  auto_seed=2443079021  user_seed=0  Tdevice=25 degC  alpha=3.93e-3 1/K  Tmeas=25 degC  thermal_mass=100 J/K  power_derating_T1=70 degC  power_derating_T2=155 degC  operating_temperature_range_vec=[-50, 150] degC  temperature_specify=off  temperature_priority=High  temperature=298.15 K  temperature_nominal_specify=off  temperature_nominal_unit=K  temperature_nominal_value=1
  Resistor12 : ee_lib/Passive/Resistor  R=0.5 kOhm  R_tol=5  enable_R_tol=0  tol_distribution=1  nSigma=4  enable_operating_limits=0  operating_limit_action=2  max_working_voltage=100 V  power_rating=1 W  enable_faults=0  fault_action=1  R_faulted=inf Ohm  enable_temporal_fault=0  t_fault=1 s  enable_behavioral_fault=0  max_permissible_current=1 A  t_fail_on_current=1 s  noise_mode=0  sample_time=1e-3 s  repeatability=1  auto_seed=2016017452  user_seed=0  Tdevice=25 degC  alpha=3.93e-3 1/K  Tmeas=25 degC  thermal_mass=100 J/K  power_derating_T1=70 degC  power_derating_T2=155 degC  operating_temperature_range_vec=[-50, 150] degC  temperature_specify=off  temperature_priority=High  temperature=298.15 K  temperature_nominal_specify=off  temperature_nominal_unit=K  temperature_nominal_value=1
  Resistor13 : ee_lib/Passive/Resistor  R=0.005 kOhm  R_tol=5  enable_R_tol=0  tol_distribution=1  nSigma=4  enable_operating_limits=0  operating_limit_action=2  max_working_voltage=100 V  power_rating=1 W  enable_faults=0  fault_action=1  R_faulted=inf Ohm  enable_temporal_fault=0  t_fault=1 s  enable_behavioral_fault=0  max_permissible_current=1 A  t_fail_on_current=1 s  noise_mode=0  sample_time=1e-3 s  repeatability=1  auto_seed=51119000  user_seed=0  Tdevice=25 degC  alpha=3.93e-3 1/K  Tmeas=25 degC  thermal_mass=100 J/K  power_derating_T1=70 degC  power_derating_T2=155 degC  operating_temperature_range_vec=[-50, 150] degC  temperature_specify=off  temperature_priority=High  temperature=298.15 K  temperature_nominal_specify=off  temperature_nominal_unit=K  temperature_nominal_value=1
  Resistor14 : ee_lib/Passive/Resistor  R=5 kOhm  R_tol=5  enable_R_tol=0  tol_distribution=1  nSigma=4  enable_operating_limits=0  operating_limit_action=2  max_working_voltage=100 V  power_rating=1 W  enable_faults=0  fault_action=1  R_faulted=inf Ohm  enable_temporal_fault=0  t_fault=1 s  enable_behavioral_fault=0  max_permissible_current=1 A  t_fail_on_current=1 s  noise_mode=0  sample_time=1e-3 s  repeatability=1  auto_seed=1447930733  user_seed=0  Tdevice=25 degC  alpha=3.93e-3 1/K  Tmeas=25 degC  thermal_mass=100 J/K  power_derating_T1=70 degC  power_derating_T2=155 degC  operating_temperature_range_vec=[-50, 150] degC  temperature_specify=off  temperature_priority=High  temperature=298.15 K  temperature_nominal_specify=off  temperature_nominal_unit=K  temperature_nominal_value=1
  Resistor15 : ee_lib/Passive/Resistor  Commented=on  R=0.7 kOhm  R_tol=5  enable_R_tol=0  tol_distribution=1  nSigma=4  enable_operating_limits=0  operating_limit_action=2  max_working_voltage=100 V  power_rating=1 W  enable_faults=0  fault_action=1  R_faulted=inf Ohm  enable_temporal_fault=0  t_fault=1 s  enable_behavioral_fault=0  max_permissible_current=1 A  t_fail_on_current=1 s  noise_mode=0  sample_time=1e-3 s  repeatability=1  auto_seed=1766665933  user_seed=0  Tdevice=25 degC  alpha=3.93e-3 1/K  Tmeas=25 degC  thermal_mass=100 J/K  power_derating_T1=70 degC  power_derating_T2=155 degC  operating_temperature_range_vec=[-50, 150] degC  temperature_specify=off  temperature_priority=High  temperature=298.15 K  temperature_nominal_specify=off  temperature_nominal_unit=K  temperature_nominal_value=1
  Resistor16 : ee_lib/Passive/Resistor  Commented=on  R=0.01 kOhm  R_tol=5  enable_R_tol=0  tol_distribution=1  nSigma=4  enable_operating_limits=0  operating_limit_action=2  max_working_voltage=100 V  power_rating=1 W  enable_faults=0  fault_action=1  R_faulted=inf Ohm  enable_temporal_fault=0  t_fault=1 s  enable_behavioral_fault=0  max_permissible_current=1 A  t_fail_on_current=1 s  noise_mode=0  sample_time=1e-3 s  repeatability=1  auto_seed=2742721817  user_seed=0  Tdevice=25 degC  alpha=3.93e-3 1/K  Tmeas=25 degC  thermal_mass=100 J/K  power_derating_T1=70 degC  power_derating_T2=155 degC  operating_temperature_range_vec=[-50, 150] degC  temperature_specify=off  temperature_priority=High  temperature=298.15 K  temperature_nominal_specify=off  temperature_nominal_unit=K  temperature_nominal_value=1
  Resistor17 : ee_lib/Passive/Resistor  Commented=on  R=0.3 kOhm  R_tol=5  enable_R_tol=0  tol_distribution=1  nSigma=4  enable_operating_limits=0  operating_limit_action=2  max_working_voltage=100 V  power_rating=1 W  enable_faults=0  fault_action=1  R_faulted=inf Ohm  enable_temporal_fault=0  t_fault=1 s  enable_behavioral_fault=0  max_permissible_current=1 A  t_fail_on_current=1 s  noise_mode=0  sample_time=1e-3 s  repeatability=1  auto_seed=3678884142  user_seed=0  Tdevice=25 degC  alpha=3.93e-3 1/K  Tmeas=25 degC  thermal_mass=100 J/K  power_derating_T1=70 degC  power_derating_T2=155 degC  operating_temperature_range_vec=[-50, 150] degC  temperature_specify=off  temperature_priority=High  temperature=298.15 K  temperature_nominal_specify=off  temperature_nominal_unit=K  temperature_nominal_value=1
  Resistor18 : ee_lib/Passive/Resistor  Commented=on  R=0.005 kOhm  R_tol=5  enable_R_tol=0  tol_distribution=1  nSigma=4  enable_operating_limits=0  operating_limit_action=2  max_working_voltage=100 V  power_rating=1 W  enable_faults=0  fault_action=1  R_faulted=inf Ohm  enable_temporal_fault=0  t_fault=1 s  enable_behavioral_fault=0  max_permissible_current=1 A  t_fail_on_current=1 s  noise_mode=0  sample_time=1e-3 s  repeatability=1  auto_seed=3279529794  user_seed=0  Tdevice=25 degC  alpha=3.93e-3 1/K  Tmeas=25 degC  thermal_mass=100 J/K  power_derating_T1=70 degC  power_derating_T2=155 degC  operating_temperature_range_vec=[-50, 150] degC  temperature_specify=off  temperature_priority=High  temperature=298.15 K  temperature_nominal_specify=off  temperature_nominal_unit=K  temperature_nominal_value=1
  Resistor19 : ee_lib/Passive/Resistor  Commented=on  R=0.5 kOhm  R_tol=5  enable_R_tol=0  tol_distribution=1  nSigma=4  enable_operating_limits=0  operating_limit_action=2  max_working_voltage=100 V  power_rating=1 W  enable_faults=0  fault_action=1  R_faulted=inf Ohm  enable_temporal_fault=0  t_fault=1 s  enable_behavioral_fault=0  max_permissible_current=1 A  t_fail_on_current=1 s  noise_mode=0  sample_time=1e-3 s  repeatability=1  auto_seed=4192576547  user_seed=0  Tdevice=25 degC  alpha=3.93e-3 1/K  Tmeas=25 degC  thermal_mass=100 J/K  power_derating_T1=70 degC  power_derating_T2=155 degC  operating_temperature_range_vec=[-50, 150] degC  temperature_specify=off  temperature_priority=High  temperature=298.15 K  temperature_nominal_specify=off  temperature_nominal_unit=K  temperature_nominal_value=1
  Resistor20 : ee_lib/Passive/Resistor  R=0.7 kOhm  R_tol=5  enable_R_tol=0  tol_distribution=1  nSigma=4  enable_operating_limits=0  operating_limit_action=2  max_working_voltage=100 V  power_rating=1 W  enable_faults=0  fault_action=1  R_faulted=inf Ohm  enable_temporal_fault=0  t_fault=1 s  enable_behavioral_fault=0  max_permissible_current=1 A  t_fail_on_current=1 s  noise_mode=0  sample_time=1e-3 s  repeatability=1  auto_seed=557942917  user_seed=0  Tdevice=25 degC  alpha=3.93e-3 1/K  Tmeas=25 degC  thermal_mass=100 J/K  power_derating_T1=70 degC  power_derating_T2=155 degC  operating_temperature_range_vec=[-50, 150] degC  temperature_specify=off  temperature_priority=High  temperature=298.15 K  temperature_nominal_specify=off  temperature_nominal_unit=K  temperature_nominal_value=1
  Resistor21 : ee_lib/Passive/Resistor  R=0.01 kOhm  R_tol=5  enable_R_tol=0  tol_distribution=1  nSigma=4  enable_operating_limits=0  operating_limit_action=2  max_working_voltage=100 V  power_rating=1 W  enable_faults=0  fault_action=1  R_faulted=inf Ohm  enable_temporal_fault=0  t_fault=1 s  enable_behavioral_fault=0  max_permissible_current=1 A  t_fail_on_current=1 s  noise_mode=0  sample_time=1e-3 s  repeatability=1  auto_seed=2443079021  user_seed=0  Tdevice=25 degC  alpha=3.93e-3 1/K  Tmeas=25 degC  thermal_mass=100 J/K  power_derating_T1=70 degC  power_derating_T2=155 degC  operating_temperature_range_vec=[-50, 150] degC  temperature_specify=off  temperature_priority=High  temperature=298.15 K  temperature_nominal_specify=off  temperature_nominal_unit=K  temperature_nominal_value=1
  Resistor22 : ee_lib/Passive/Resistor  R=0.5 kOhm  R_tol=5  enable_R_tol=0  tol_distribution=1  nSigma=4  enable_operating_limits=0  operating_limit_action=2  max_working_voltage=100 V  power_rating=1 W  enable_faults=0  fault_action=1  R_faulted=inf Ohm  enable_temporal_fault=0  t_fault=1 s  enable_behavioral_fault=0  max_permissible_current=1 A  t_fail_on_current=1 s  noise_mode=0  sample_time=1e-3 s  repeatability=1  auto_seed=2016017452  user_seed=0  Tdevice=25 degC  alpha=3.93e-3 1/K  Tmeas=25 degC  thermal_mass=100 J/K  power_derating_T1=70 degC  power_derating_T2=155 degC  operating_temperature_range_vec=[-50, 150] degC  temperature_specify=off  temperature_priority=High  temperature=298.15 K  temperature_nominal_specify=off  temperature_nominal_unit=K  temperature_nominal_value=1
  Resistor23 : ee_lib/Passive/Resistor  R=0.005 kOhm  R_tol=5  enable_R_tol=0  tol_distribution=1  nSigma=4  enable_operating_limits=0  operating_limit_action=2  max_working_voltage=100 V  power_rating=1 W  enable_faults=0  fault_action=1  R_faulted=inf Ohm  enable_temporal_fault=0  t_fault=1 s  enable_behavioral_fault=0  max_permissible_current=1 A  t_fail_on_current=1 s  noise_mode=0  sample_time=1e-3 s  repeatability=1  auto_seed=51119000  user_seed=0  Tdevice=25 degC  alpha=3.93e-3 1/K  Tmeas=25 degC  thermal_mass=100 J/K  power_derating_T1=70 degC  power_derating_T2=155 degC  operating_temperature_range_vec=[-50, 150] degC  temperature_specify=off  temperature_priority=High  temperature=298.15 K  temperature_nominal_specify=off  temperature_nominal_unit=K  temperature_nominal_value=1
  Resistor24 : ee_lib/Passive/Resistor  R=5 kOhm  R_tol=5  enable_R_tol=0  tol_distribution=1  nSigma=4  enable_operating_limits=0  operating_limit_action=2  max_working_voltage=100 V  power_rating=1 W  enable_faults=0  fault_action=1  R_faulted=inf Ohm  enable_temporal_fault=0  t_fault=1 s  enable_behavioral_fault=0  max_permissible_current=1 A  t_fail_on_current=1 s  noise_mode=0  sample_time=1e-3 s  repeatability=1  auto_seed=1447930733  user_seed=0  Tdevice=25 degC  alpha=3.93e-3 1/K  Tmeas=25 degC  thermal_mass=100 J/K  power_derating_T1=70 degC  power_derating_T2=155 degC  operating_temperature_range_vec=[-50, 150] degC  temperature_specify=off  temperature_priority=High  temperature=298.15 K  temperature_nominal_specify=off  temperature_nominal_unit=K  temperature_nominal_value=1
  Resistor5 : ee_lib/Passive/Resistor  Commented=on  R=0.5 kOhm  R_tol=5  enable_R_tol=0  tol_distribution=1  nSigma=4  enable_operating_limits=0  operating_limit_action=2  max_working_voltage=100 V  power_rating=1 W  enable_faults=0  fault_action=1  R_faulted=inf Ohm  enable_temporal_fault=0  t_fault=1 s  enable_behavioral_fault=0  max_permissible_current=1 A  t_fail_on_current=1 s  noise_mode=0  sample_time=1e-3 s  repeatability=1  auto_seed=2257268386  user_seed=0  Tdevice=25 degC  alpha=3.93e-3 1/K  Tmeas=25 degC  thermal_mass=100 J/K  power_derating_T1=70 degC  power_derating_T2=155 degC  operating_temperature_range_vec=[-50, 150] degC  temperature_specify=off  temperature_priority=High  temperature=298.15 K  temperature_nominal_specify=off  temperature_nominal_unit=K  temperature_nominal_value=1
  Resistor6 : ee_lib/Passive/Resistor  Commented=on  R=0.01 kOhm  R_tol=5  enable_R_tol=0  tol_distribution=1  nSigma=4  enable_operating_limits=0  operating_limit_action=2  max_working_voltage=100 V  power_rating=1 W  enable_faults=0  fault_action=1  R_faulted=inf Ohm  enable_temporal_fault=0  t_fault=1 s  enable_behavioral_fault=0  max_permissible_current=1 A  t_fail_on_current=1 s  noise_mode=0  sample_time=1e-3 s  repeatability=1  auto_seed=1115072639  user_seed=0  Tdevice=25 degC  alpha=3.93e-3 1/K  Tmeas=25 degC  thermal_mass=100 J/K  power_derating_T1=70 degC  power_derating_T2=155 degC  operating_temperature_range_vec=[-50, 150] degC  temperature_specify=off  temperature_priority=High  temperature=298.15 K  temperature_nominal_specify=off  temperature_nominal_unit=K  temperature_nominal_value=1
  Resistor7 : ee_lib/Passive/Resistor  Commented=on  R=5 kOhm  R_tol=5  enable_R_tol=0  tol_distribution=1  nSigma=4  enable_operating_limits=0  operating_limit_action=2  max_working_voltage=100 V  power_rating=1 W  enable_faults=0  fault_action=1  R_faulted=inf Ohm  enable_temporal_fault=0  t_fault=1 s  enable_behavioral_fault=0  max_permissible_current=1 A  t_fail_on_current=1 s  noise_mode=0  sample_time=1e-3 s  repeatability=1  auto_seed=219777202  user_seed=0  Tdevice=25 degC  alpha=3.93e-3 1/K  Tmeas=25 degC  thermal_mass=100 J/K  power_derating_T1=70 degC  power_derating_T2=155 degC  operating_temperature_range_vec=[-50, 150] degC  temperature_specify=off  temperature_priority=High  temperature=298.15 K  temperature_nominal_specify=off  temperature_nominal_unit=K  temperature_nominal_value=1
  Resistor8 : ee_lib/Passive/Resistor  Commented=on  R=0.005 kOhm  R_tol=5  enable_R_tol=0  tol_distribution=1  nSigma=4  enable_operating_limits=0  operating_limit_action=2  max_working_voltage=100 V  power_rating=1 W  enable_faults=0  fault_action=1  R_faulted=inf Ohm  enable_temporal_fault=0  t_fault=1 s  enable_behavioral_fault=0  max_permissible_current=1 A  t_fail_on_current=1 s  noise_mode=0  sample_time=1e-3 s  repeatability=1  auto_seed=3143701867  user_seed=0  Tdevice=25 degC  alpha=3.93e-3 1/K  Tmeas=25 degC  thermal_mass=100 J/K  power_derating_T1=70 degC  power_derating_T2=155 degC  operating_temperature_range_vec=[-50, 150] degC  temperature_specify=off  temperature_priority=High  temperature=298.15 K  temperature_nominal_specify=off  temperature_nominal_unit=K  temperature_nominal_value=1
  Resistor9 : ee_lib/Passive/Resistor  Commented=on  R=5 kOhm  R_tol=5  enable_R_tol=0  tol_distribution=1  nSigma=4  enable_operating_limits=0  operating_limit_action=2  max_working_voltage=100 V  power_rating=1 W  enable_faults=0  fault_action=1  R_faulted=inf Ohm  enable_temporal_fault=0  t_fault=1 s  enable_behavioral_fault=0  max_permissible_current=1 A  t_fail_on_current=1 s  noise_mode=0  sample_time=1e-3 s  repeatability=1  auto_seed=705626151  user_seed=0  Tdevice=25 degC  alpha=3.93e-3 1/K  Tmeas=25 degC  thermal_mass=100 J/K  power_derating_T1=70 degC  power_derating_T2=155 degC  operating_temperature_range_vec=[-50, 150] degC  temperature_specify=off  temperature_priority=High  temperature=298.15 K  temperature_nominal_specify=off  temperature_nominal_unit=K  temperature_nominal_value=1
  Scope{6,8,10..12,19..23} (10 alike) : Scope  Commented=on
  Scope{13..17,25..26,28..30} (10 alike) : Scope
  Scope18 : Scope  NumInputPorts=2
  Scope24 : Scope  Commented=on  NumInputPorts=2
  Scope27 : Scope  NumInputPorts=2
  Scope9 : Scope  Commented=on  NumInputPorts=2
  Simulink-PS Converter{5..6,9..10} (4 alike) : nesl_utility/Simulink-PS Converter  PhysicalDomain=network_engine_domain  SubClassName=ps_input  LeftPortType=input  RightPortType=output  PseudoPeriodic=off  Frequencies=[]  NoiseDistribution=none  NoiseParameters=[]  Unit=1  AffineConversion=off  FilteringAndDerivatives=provide  SimscapeFilterOrder=1  InputFilterTimeConstant=0.001  UdotUserProvided=0
      settings: SourceProductBaseCode=PW,SS
  Simulink-PS Converter{2,4,7..8} (4 alike) : nesl_utility/Simulink-PS Converter  Commented=on  PhysicalDomain=network_engine_domain  SubClassName=ps_input  LeftPortType=input  RightPortType=output  PseudoPeriodic=off  Frequencies=[]  NoiseDistribution=none  NoiseParameters=[]  Unit=1  AffineConversion=off  FilteringAndDerivatives=provide  SimscapeFilterOrder=1  InputFilterTimeConstant=0.001  UdotUserProvided=0
      settings: SourceProductBaseCode=PW,SS
  Solver Configuration1 : nesl_utility/Solver Configuration  Commented=on  PhysicalDomain=network_engine_domain  SubClassName=solver  LeftPortType=input  RightPortType=generic  Tones=[]  Harmonics=[]  SimulateNoise=off  Profile=off  UseLocalSampling=off  EnableSwitchedLinearOptims=on  FrequencyDomain=off  UseCCode=off  RelTol=0.001  AbsTol=1e-06  MinStep=1e-09  ToWorkspace=off  RevertToSquareIcSolve=off  NumHomotopyIterations=100  PhasorMode=off  PhasorModeNumHarmonics=1  DoDC=off  ResidualTolerance=1e-09  UseLocalSolver=off  LocalSolverChoice=NE_BACKWARD_EULER_ADVANCER  LocalSolverSampleTime=0.001  DoFixedCost=off  MaxNonlinIter=3  MaxModeIter=2  ComputeImpulses=off  ImpulseIterations=2  LinearAlgebra=auto  EquationFormulation=NE_TIME_EF  DelaysMemoryBudget=1024  AutomaticFiltering=on  FilteringTimeConstant=0.001  PartitionStorageMethod=AS_NEEDED  PartitionMemoryBudget=1024  PartitionMethod=ROBUST
      settings: SourceProductBaseCode=PW,SS
  Solver Configuration2 : nesl_utility/Solver Configuration  PhysicalDomain=network_engine_domain  SubClassName=solver  LeftPortType=input  RightPortType=generic  Tones=[]  Harmonics=[]  SimulateNoise=off  Profile=off  UseLocalSampling=off  EnableSwitchedLinearOptims=on  FrequencyDomain=off  UseCCode=off  RelTol=0.001  AbsTol=1e-06  MinStep=1e-09  ToWorkspace=off  RevertToSquareIcSolve=off  NumHomotopyIterations=100  PhasorMode=off  PhasorModeNumHarmonics=1  DoDC=off  ResidualTolerance=1e-09  UseLocalSolver=off  LocalSolverChoice=NE_BACKWARD_EULER_ADVANCER  LocalSolverSampleTime=0.001  DoFixedCost=off  MaxNonlinIter=3  MaxModeIter=2  ComputeImpulses=off  ImpulseIterations=2  LinearAlgebra=auto  EquationFormulation=NE_TIME_EF  DelaysMemoryBudget=1024  AutomaticFiltering=on  FilteringTimeConstant=0.001  PartitionStorageMethod=AS_NEEDED  PartitionMemoryBudget=1024  PartitionMethod=ROBUST
      settings: SourceProductBaseCode=PW,SS
  Solver Configuration3 : nesl_utility/Solver Configuration  Commented=on  PhysicalDomain=network_engine_domain  SubClassName=solver  LeftPortType=input  RightPortType=generic  Tones=[]  Harmonics=[]  SimulateNoise=off  Profile=off  UseLocalSampling=off  EnableSwitchedLinearOptims=on  FrequencyDomain=off  UseCCode=off  RelTol=0.001  AbsTol=1e-06  MinStep=1e-09  ToWorkspace=off  RevertToSquareIcSolve=off  NumHomotopyIterations=100  PhasorMode=off  PhasorModeNumHarmonics=1  DoDC=off  ResidualTolerance=1e-09  UseLocalSolver=off  LocalSolverChoice=NE_BACKWARD_EULER_ADVANCER  LocalSolverSampleTime=0.001  DoFixedCost=off  MaxNonlinIter=3  MaxModeIter=2  ComputeImpulses=off  ImpulseIterations=2  LinearAlgebra=auto  EquationFormulation=NE_TIME_EF  DelaysMemoryBudget=1024  AutomaticFiltering=on  FilteringTimeConstant=0.001  PartitionStorageMethod=AS_NEEDED  PartitionMemoryBudget=1024  PartitionMethod=ROBUST
      settings: SourceProductBaseCode=PW,SS
  Solver Configuration4 : nesl_utility/Solver Configuration  PhysicalDomain=network_engine_domain  SubClassName=solver  LeftPortType=input  RightPortType=generic  Tones=[]  Harmonics=[]  SimulateNoise=off  Profile=off  UseLocalSampling=off  EnableSwitchedLinearOptims=on  FrequencyDomain=off  UseCCode=off  RelTol=0.001  AbsTol=1e-06  MinStep=1e-09  ToWorkspace=off  RevertToSquareIcSolve=off  NumHomotopyIterations=100  PhasorMode=off  PhasorModeNumHarmonics=1  DoDC=off  ResidualTolerance=1e-09  UseLocalSolver=off  LocalSolverChoice=NE_BACKWARD_EULER_ADVANCER  LocalSolverSampleTime=0.001  DoFixedCost=off  MaxNonlinIter=3  MaxModeIter=2  ComputeImpulses=off  ImpulseIterations=2  LinearAlgebra=auto  EquationFormulation=NE_TIME_EF  DelaysMemoryBudget=1024  AutomaticFiltering=on  FilteringTimeConstant=0.001  PartitionStorageMethod=AS_NEEDED  PartitionMemoryBudget=1024  PartitionMethod=ROBUST
      settings: SourceProductBaseCode=PW,SS
  Subsystem1 : Subsystem  Commented=on
      settings: PortSchema="{\"entries\":[{\"content\":{\"sides\":[{\"content\":{\"connectorIds\":[\"Out2\"]},\"type\":\"ConnectorPlacement.EquallySpacedRectSide\",\"uuid\":\"03ba92a8-40e6-4801-8309-99fae415c558\"},{\"content\":{\"connectorIds\":[\"Out1\"],\"side\":\"RIGHT\"},\"type\":\"ConnectorPlacement.EquallySpacedRectSide\",\"uuid\":\"ac43c488-4010-4e11-8920-21da616a0e9d\"},{\"content\":{\"connectorIds\":[],\"side\":\"TOP\"},\"type\":\"ConnectorPlacement.EquallySpacedRectSide\",\"uuid\":\"57f88e2e-9b42-4ae1-8038-2365f967330a\"}]},\"type\":\"ConnectorPlacement.EquallySpacedConnector\",\"uuid\":\"ba10684c-0747-4aa3-97a0-f43249d9425c\"}],\"packageUris\":[\"http://schema.mathworks.com/mf0/Connector/R2020b\"],\"version\":\"1.0\"}"
  Subsystem3 : Subsystem
      settings: PortSchema="{\"entries\":[{\"content\":{\"sides\":[{\"content\":{\"connectorIds\":[\"Out2\"]},\"type\":\"ConnectorPlacement.EquallySpacedRectSide\",\"uuid\":\"03ba92a8-40e6-4801-8309-99fae415c558\"},{\"content\":{\"connectorIds\":[\"Out1\"],\"side\":\"RIGHT\"},\"type\":\"ConnectorPlacement.EquallySpacedRectSide\",\"uuid\":\"ac43c488-4010-4e11-8920-21da616a0e9d\"},{\"content\":{\"connectorIds\":[],\"side\":\"TOP\"},\"type\":\"ConnectorPlacement.EquallySpacedRectSide\",\"uuid\":\"57f88e2e-9b42-4ae1-8038-2365f967330a\"}]},\"type\":\"ConnectorPlacement.EquallySpacedConnector\",\"uuid\":\"ba10684c-0747-4aa3-97a0-f43249d9425c\"}],\"packageUris\":[\"http://schema.mathworks.com/mf0/Connector/R2020b\"],\"version\":\"1.0\"}"
  Subsystem4 : Subsystem  Commented=on
      settings: PortSchema="{\"entries\":[{\"content\":{\"sides\":[{\"content\":{\"connectorIds\":[\"Out2\"]},\"type\":\"ConnectorPlacement.EquallySpacedRectSide\",\"uuid\":\"03ba92a8-40e6-4801-8309-99fae415c558\"},{\"content\":{\"connectorIds\":[\"Out1\"],\"side\":\"RIGHT\"},\"type\":\"ConnectorPlacement.EquallySpacedRectSide\",\"uuid\":\"ac43c488-4010-4e11-8920-21da616a0e9d\"},{\"content\":{\"connectorIds\":[],\"side\":\"TOP\"},\"type\":\"ConnectorPlacement.EquallySpacedRectSide\",\"uuid\":\"57f88e2e-9b42-4ae1-8038-2365f967330a\"}]},\"type\":\"ConnectorPlacement.EquallySpacedConnector\",\"uuid\":\"ba10684c-0747-4aa3-97a0-f43249d9425c\"}],\"packageUris\":[\"http://schema.mathworks.com/mf0/Connector/R2020b\"],\"version\":\"1.0\"}"
  Subsystem5 : Subsystem
      settings: PortSchema="{\"entries\":[{\"content\":{\"sides\":[{\"content\":{\"connectorIds\":[\"Out2\"]},\"type\":\"ConnectorPlacement.EquallySpacedRectSide\",\"uuid\":\"03ba92a8-40e6-4801-8309-99fae415c558\"},{\"content\":{\"connectorIds\":[\"Out1\"],\"side\":\"RIGHT\"},\"type\":\"ConnectorPlacement.EquallySpacedRectSide\",\"uuid\":\"ac43c488-4010-4e11-8920-21da616a0e9d\"},{\"content\":{\"connectorIds\":[],\"side\":\"TOP\"},\"type\":\"ConnectorPlacement.EquallySpacedRectSide\",\"uuid\":\"57f88e2e-9b42-4ae1-8038-2365f967330a\"}]},\"type\":\"ConnectorPlacement.EquallySpacedConnector\",\"uuid\":\"ba10684c-0747-4aa3-97a0-f43249d9425c\"}],\"packageUris\":[\"http://schema.mathworks.com/mf0/Connector/R2020b\"],\"version\":\"1.0\"}"
  To Workspace1 : ToWorkspace  Commented=on  VariableName=AorticStenosis  SaveFormat=Timeseries  SampleTime=-1
  To Workspace2 : ToWorkspace  VariableName=H  SaveFormat=Timeseries  SampleTime=-1
  To Workspace3 : ToWorkspace  VariableName=NormalAorta1  SaveFormat=Timeseries  SampleTime=-1
  Tricuspid Valve1 : fl_lib/Electrical/Electrical Elements/Diode  Commented=on  Vf=0.6 V  Ron=0.03 Ohm  Goff=1e-8 1/Ohm  i_specify=off  i_priority=None  i=0 A  i_nominal_specify=off  i_nominal_unit=A  i_nominal_value=1  v_specify=off  v_priority=None  v=0 V  v_nominal_specify=off  v_nominal_unit=V  v_nominal_value=1
  Tricuspid Valve2 : fl_lib/Electrical/Electrical Elements/Diode  Vf=0.6 V  Ron=0.03 Ohm  Goff=1e-8 1/Ohm  i_specify=off  i_priority=None  i=0 A  i_nominal_specify=off  i_nominal_unit=A  i_nominal_value=1  v_specify=off  v_priority=None  v=0 V  v_nominal_specify=off  v_nominal_unit=V  v_nominal_value=1
  Tricuspid Valve3 : fl_lib/Electrical/Electrical Elements/Diode  Commented=on  Vf=0.6 V  Ron=0.03 Ohm  Goff=1e-8 1/Ohm  i_specify=off  i_priority=None  i=0 A  i_nominal_specify=off  i_nominal_unit=A  i_nominal_value=1  v_specify=off  v_priority=None  v=0 V  v_nominal_specify=off  v_nominal_unit=V  v_nominal_value=1
  Tricuspid Valve4 : fl_lib/Electrical/Electrical Elements/Diode  Vf=0.6 V  Ron=0.03 Ohm  Goff=1e-8 1/Ohm  i_specify=off  i_priority=None  i=0 A  i_nominal_specify=off  i_nominal_unit=A  i_nominal_value=1  v_specify=off  v_priority=None  v=0 V  v_nominal_specify=off  v_nominal_unit=V  v_nominal_value=1
  Voltage Sensor{5,7..10,16..20} (10 alike) : fl_lib/Electrical/Electrical Sensors/Voltage Sensor  Commented=on
  Voltage Sensor{11..15,21..25} (10 alike) : fl_lib/Electrical/Electrical Sensors/Voltage Sensor
  wires:
  Subsystem1/2(Out2) -> Simulink-PS Converter4/1
  PS-Simulink Converter9/1 -> Scope11/1
  PS-Simulink Converter8/1 -> Scope10/1
  PS-Simulink Converter10/1 -> Scope12/1
  Subsystem1/1(Out1) -> Simulink-PS Converter2/1
  PS-Simulink Converter7/1 -> Scope9/2, To Workspace1/1, Scope8/1
  PS-Simulink Converter5/1 -> Scope9/1, Scope6/1
  PS-Simulink Converter12/1 -> Scope16/1, Scope18/1
  PS-Simulink Converter13/1 -> Scope17/1, To Workspace2/1, Scope18/2
  Subsystem3/1(Out1) -> Simulink-PS Converter5/1
  PS-Simulink Converter11/1 -> Scope15/1
  PS-Simulink Converter14/1 -> Scope13/1
  PS-Simulink Converter15/1 -> Scope14/1
  Subsystem3/2(Out2) -> Simulink-PS Converter6/1
  PS-Simulink Converter19/1 -> Scope19/1
  PS-Simulink Converter17/1 -> Scope22/1, Scope24/1
  Subsystem4/2(Out2) -> Simulink-PS Converter8/1
  PS-Simulink Converter16/1 -> Scope21/1
  PS-Simulink Converter18/1 -> Scope23/1, Scope24/2
  PS-Simulink Converter20/1 -> Scope20/1
  Subsystem4/1(Out1) -> Simulink-PS Converter7/1
  Subsystem5/2(Out2) -> Simulink-PS Converter10/1
  Subsystem5/1(Out1) -> Simulink-PS Converter9/1
  PS-Simulink Converter24/1 -> Scope29/1
  PS-Simulink Converter22/1 -> Scope26/1, To Workspace3/1, Scope27/2
  PS-Simulink Converter23/1 -> Scope28/1
  PS-Simulink Converter21/1 -> Scope25/1, Scope27/1
  PS-Simulink Converter25/1 -> Scope30/1
  connections:
  C-BrachiocephalicArtery1/LConn1 -- L1/LConn1 -- L-BrachiocephalicArtery1/RConn1
  C-Ulnar Artery3/LConn1 -- L-Ulnar Artery3/RConn1 -- C-Radial Artery3/LConn1 -- L-Radial Artery3/RConn1 -- R- R Brachial1/LConn1
  R- Right Internal Carotid1/LConn1 -- R- Right External Carotid1/LConn1 -- R-Ulnar Artery3/LConn1 -- Voltage Sensor10/LConn1 -- R-Rdial Artery3/LConn1
  C- Splentic1/LConn1 -- L-Splentic1/RConn1 -- C- Left Gastric Artery1/LConn1 -- L-Left Gastric Artery1/RConn1 -- C- Right Gastric Artery1/LConn1 -- L- Right Gastric Artery1/RConn1 -- L-  Hepatic Artery1/RConn1 -- C- Hepatic Artery1/LConn1 -- C- Abdominal Aorta 2/LConn1 -- L-  Abdominal Aorta 2/RConn1 -- R-Right Common Iliac1/LConn1 -- R-Left Common Iliac1/LConn1 -- L-Inferior Mesentric1/RConn1 -- C- Inferior Mesentric1/LConn1 -- L-Superior Mesentric1/RConn1 -- C- Superior Mesentric1/LConn1 -- L-Right Renal Artery1/RConn1 -- C- Right Renal Artery1/LConn1 -- L- Left Renal Artery1/RConn1 -- C-  Left Renal Artery1/LConn1
  R- Superior Vena Cava4/LConn1 -- R- Vertebral Artery1/LConn1 -- L-Left Vertebral1/RConn1 -- C-Left Vertebral1/LConn1 -- L-Ulnar Artery2/RConn1 -- C-Ulnar Artery2/LConn1 -- Voltage Sensor8/LConn1 -- C-Radial Artery2/LConn1 -- L-Radial Artery2/RConn1
  R-RIPV1/LConn1 -- R- RSPV1/LConn1 -- C- RPA1/LConn1 -- L- RPA1/RConn1
  Solver Configuration1/RConn1 -- R-Right Pulmonary Artery1/LConn1 -- R- left Pulmonary Artery1/LConn1 -- Voltage Sensor9/LConn1 -- L- main Pulmonary Artery1/RConn1 -- C- main Pulmonary Artery1/LConn1
  Capacitor5/LConn1 -- Inductor5/RConn1 -- L-1/LConn1 -- R- Descending Aorta1/LConn1
  R- Axillary1/LConn1 -- C-Left Subcalvin2/LConn1 -- L-Left Subcalvin2/RConn1
  L- Right Ventricle1/RConn1 -- C- Right Ventricle1/LConn1 -- Pulmonary Valve1/LConn1
  R- Brachial1/LConn1 -- C-Axilary1/LConn1 -- L-Axillary1/RConn1
  L -LIPV1/RConn1 -- C-LIPV1/LConn1 -- C- LSPV1/LConn1 -- L-LSPV1/RConn1 -- C- RSPV1/LConn1 -- L- RSPV1/RConn1 -- L- RIPV1/RConn1 -- C- RIPV1/LConn1 -- R- Left Atrium1/LConn1
  Voltage Sensor5/LConn1 -- Diode1/LConn1 -- Capacitor3/LConn1 -- Inductor3/RConn1
  C-Right Common Iliac1/LConn1 -- L-Right Common Iliac1/RConn1 -- R-Right External Iliac1/LConn1
  C- Left Atrium1/LConn1 -- L- Left Atrium1/RConn1 -- Mitral Valve1/LConn1
  L-Right External Carotid1/RConn1 -- C-Right External Carotid1/LConn1 -- R- Right Common Carotid A 1/LConn1 -- C-Right Internal Carotid1/LConn1 -- L-Right Internal Carotid1/RConn1
  L- Inferior Vena Cava1/RConn1 -- C- Superoir Vena Cava1/LConn1 -- L- Superior Vena Cava1/RConn1 -- R- Right Atrium1/LConn1 -- C- Inferior Vena Cava1/LConn1
  L-1/RConn1 -- R- Left Subcalvin 2/LConn1 -- R- Left Vertebral1/LConn1
  C-Vertebral Artery1/LConn1 -- L-Vertebral Artery1/RConn1 -- C-Right Common Carotid A1/LConn1 -- L-Right Common Carotid A1/RConn1 -- R- BrachiocephalicArtery1/LConn1 -- L-Right Subclavin1/RConn1 -- C-Right Subclavin1/LConn1
  Inductor4/RConn1 -- Capacitor4/LConn1 -- Voltage Sensor7/LConn1 -- Resistor6/LConn1 -- L1/RConn1
  L-Right Femoral Artery1/RConn1 -- C-Right Femoral Artery1/LConn1 -- R-L Anterior Tibial Artery1/LConn1 -- R-L Posterior Tibial Artery1/LConn1
  L- R Anterior Tibial Artery1/RConn1 -- C- Anterior Tibial Artery1/LConn1 -- L-R Posterior Tibial Artery1/RConn1 -- C- Posterior Tibial Artery1/LConn1 -- L- L Anterior Tibial Artery1/RConn1 -- C-  L Anterior Tibial Artery1/LConn1 -- L-L Posterior Tibial Artery1/RConn1 -- C- L Posterior Tibial Artery1/LConn1 -- R- Inferior Mesentric1/LConn1 -- R- Splentic1/LConn1 -- R-Left Gastric Artery1/LConn1 -- R- Hepatic Artery1/LConn1 -- R- Right Gastric Artery1/LConn1 -- R- Superior Vena Cava5/RConn1 -- R- Superior Mesentric1/LConn1 -- R- Left Renal Artery1/LConn1 -- R- Right Renal Artery1/LConn1
  C- Brachial1/LConn1 -- R-Rdial Artery2/LConn1 -- R-Ulnar Artery2/LConn1 -- L- Brachial1/RConn1
  R-LIPV1/LConn1 -- C- LPA1/LConn1 -- L- LPA1/RConn1 -- R- LSPV1/LConn1
  Mitral Valve1/RConn1 -- Resistor5/LConn1 -- DC Voltage Source1/LConn1
  R- Right Ventricle1/LConn1 -- Tricuspid Valve1/RConn1 -- DC Voltage Source4/LConn1
  L-Right External Iliac1/RConn1 -- C-Right External Iliac1/LConn1 -- R-Right Femoral Artery1/LConn1
  R-R Posterior Tibial Artery1/LConn1 -- R-R Anterior Tibial Artery1/LConn1 -- L-Left Femoral Artery1/RConn1 -- C- Left Femoral Artery1/LConn1
  C-axilary1/LConn1 -- L-axilary1/RConn1 -- R- Right Subclavin1/LConn1
  C- Left External Iliac1/LConn1 -- L-Left External Iliac1/RConn1 -- R-Left Femoral Artery1/LConn1
  L R Brachial1/RConn1 -- C- R Brachial1/LConn1 -- R- axilary1/LConn1
  C- Left Common Iliac1/LConn1 -- L-Left Common Iliac1/RConn1 -- R-Left External Iliac1/LConn1
  L- Right Atrium1/RConn1 -- C- Right Atrium1/LConn1 -- Tricuspid Valve1/LConn1
  L-  Descending Aorta1/RConn1 -- R-  Abdominal Aorta1/LConn1 -- C- Descending Aorta1/LConn1
  R- Splentic1/RConn1 -- L-Splentic1/LConn1
  R-Visco Left Gastric1/LConn1 -- C- Left Gastric Artery1/RConn1
  C- Superoir Vena Cava1/RConn1 -- Electrical Reference71/LConn1
  R- Brachial1/RConn1 -- L- Brachial1/LConn1
  Diode1/RConn1 -- Resistor7/LConn1
  R- Superior Vena Cava3/LConn1 -- R- Superior Vena Cava4/RConn1
  C- Posterior Tibial Artery1/RConn1 -- R-Visco PT1/LConn1
  Voltage Sensor10/RConn1 -- PS-Simulink Converter10/LConn1
  DC Voltage Source1/RConn1 -- Controlled Voltage Source2/LConn1
  Resistor8/LConn1 -- Capacitor5/RConn1
  R-Visco SM1/LConn1 -- C- Superior Mesentric1/RConn1
  R- visco  Brachial1/RConn1 -- Electrical Reference80/LConn1
  C- RIPV1/RConn1 -- Electrical Reference119/LConn1
  R-Rdial Artery3/RConn1 -- L-Radial Artery3/LConn1
  L R Brachial1/LConn1 -- R- R Brachial1/RConn1
  R- Right Common Carotid A 1/RConn1 -- L-Right Common Carotid A1/LConn1
  R- Hepatic Artery1/RConn1 -- L-  Hepatic Artery1/LConn1
  R-Left Femoral Artery1/RConn1 -- L-Left Femoral Artery1/LConn1
  C- LPA1/RConn1 -- R- LPA1/LConn1
  R-R Viscielastic1/RConn1 -- Electrical Reference62/LConn1
  Voltage Sensor7/RConn2 -- Electrical Reference72/LConn1
  Voltage Sensor8/RConn2 -- Electrical Reference69/LConn1
  R- L Visco AT1/RConn1 -- Electrical Reference99/LConn1
  R- visco Left Vertebral1/RConn1 -- Electrical Reference117/LConn1
  R- Left Renal Artery1/RConn1 -- L- Left Renal Artery1/LConn1
  L-  Abdominal Aorta 2/LConn1 -- R-  Abdominal Aorta1/RConn1
  L- Right Ventricle1/LConn1 -- R- Right Ventricle1/RConn1
  R- Left Subcalvin 2/RConn1 -- L-Left Subcalvin2/LConn1
  PS-Simulink Converter8/LConn1 -- Voltage Sensor8/RConn1
  L- Inferior Vena Cava1/LConn1 -- R- Inferior Vena Cava1/RConn1
  L- RPA1/LConn1 -- R-Right Pulmonary Artery1/RConn1
  C- Descending Aorta1/RConn1 -- R-Viscoelastic DA1/LConn1
  R-LIPV1/RConn1 -- L -LIPV1/LConn1
  Voltage Sensor9/RConn1 -- PS-Simulink Converter9/LConn1
  Electrical Reference76/LConn1 -- C- Inferior Vena Cava1/RConn1
  Electrical Reference75/LConn1 -- R-Viscoelastic DA1/RConn1
  R- Superior Mesentric1/RConn1 -- L-Superior Mesentric1/LConn1
  R-R Anterior Tibial Artery1/RConn1 -- L- R Anterior Tibial Artery1/LConn1
  Electrical Reference88/LConn1 -- R-Visco SM1/RConn1
  L-axilary1/LConn1 -- R- axilary1/RConn1
  Capacitor3/RConn1 -- Electrical Reference51/LConn1
  R- Right Subclavin1/RConn1 -- L-Right Subclavin1/LConn1
  C-Radial Artery3/RConn1 -- R- Radial Artery3/LConn1
  C- Inferior Mesentric1/RConn1 -- R-Visco IM1/LConn1
  Electrical Reference66/LConn1 -- R- Radial Artery2/RConn1
  C- Brachial1/RConn1 -- R- visco  Brachial1/LConn1
  C- Left Atrium1/RConn1 -- Electrical Reference95/LConn1
  C-Axilary1/RConn1 -- R- visco Axilary1/LConn1
  R- BrachiocephalicArtery1/RConn1 -- L-BrachiocephalicArtery1/LConn1
  R-  R Brachial1/RConn1 -- Electrical Reference104/LConn1
  L-Right Common Iliac1/LConn1 -- R-Right Common Iliac1/RConn1
  L-Right External Iliac1/LConn1 -- R-Right External Iliac1/RConn1
  Voltage Sensor10/RConn2 -- Electrical Reference101/LConn1
  R-Visco RR1/LConn1 -- C- Right Renal Artery1/RConn1
  C- L Posterior Tibial Artery1/RConn1 -- R-L Visco PT1/LConn1
  Resistor9/LConn1 -- Capacitor4/RConn1
  Electrical Reference63/LConn1 -- C- Right Ventricle1/RConn1
  R-Left External Iliac1/RConn1 -- L-Left External Iliac1/LConn1
  R-Visco LCI1/LConn1 -- C- Left Common Iliac1/RConn1
  Electrical Reference81/LConn1 -- R-Visco Hepatic 1/RConn1
  R-Visco LCI1/RConn1 -- Electrical Reference90/LConn1
  Controlled Voltage Source4/LConn1 -- DC Voltage Source4/RConn1
  R-L Anterior Tibial Artery1/RConn1 -- L- L Anterior Tibial Artery1/LConn1
  C-Ulnar Artery3/RConn1 -- R- Ulnar Artery3/LConn1
  R- Ulnar Artery2/RConn1 -- Electrical Reference118/LConn1
  L- RSPV1/LConn1 -- R- RSPV1/RConn1
  C-Left Vertebral1/RConn1 -- R- visco Left Vertebral1/LConn1
  R- Right Renal Artery1/RConn1 -- L-Right Renal Artery1/LConn1
  R-RIPV1/RConn1 -- L- RIPV1/LConn1
  Electrical Reference68/LConn1 -- Resistor9/RConn1
  L- main Pulmonary Artery1/LConn1 -- R- main Pulmonary Artery1/RConn1
  C-Left Subcalvin2/RConn1 -- R- visco Left Subcalvin2/LConn1
  R- Left Vertebral1/RConn1 -- L-Left Vertebral1/LConn1
  R-Visco PT1/RConn1 -- Electrical Reference98/LConn1
  Voltage Sensor5/RConn1 -- PS-Simulink Converter5/LConn1
  R-Visco Right Gastric1/LConn1 -- C- Right Gastric Artery1/RConn1
  R-Visco RCI1/RConn1 -- Electrical Reference91/LConn1
  C-Right Subclavin1/RConn1 -- R- visco RS1/LConn1
  L-L Posterior Tibial Artery1/LConn1 -- R-L Posterior Tibial Artery1/RConn1
  Electrical Reference105/LConn1 -- Resistor8/RConn1
  R- LPA1/RConn1 -- Electrical Reference106/LConn1
  R-Visco REI1/LConn1 -- C-Right External Iliac1/RConn1
  L-LSPV1/LConn1 -- R- LSPV1/RConn1
  C-Right External Carotid1/RConn1 -- R- visco REC1/LConn1
  C-Right Internal Carotid1/RConn1 -- R- visco RIC1/LConn1
  Electrical Reference121/LConn1 -- C-LIPV1/RConn1
  R- visco Axilary1/RConn1 -- Electrical Reference79/LConn1
  R- Right Atrium1/RConn1 -- L- Right Atrium1/LConn1
  C- Right Atrium1/RConn1 -- Electrical Reference70/LConn1
  Pulmonary Valve1/RConn1 -- R- main Pulmonary Artery1/LConn1
  R-L Visco PT1/RConn1 -- Electrical Reference100/LConn1
  R-Visco LFA1/RConn1 -- Electrical Reference94/LConn1
  R-Visco AT1/RConn1 -- Electrical Reference97/LConn1
  Voltage Sensor9/RConn2 -- Electrical Reference67/LConn1
  R- Viscoelastic1/RConn1 -- Electrical Reference64/LConn1
  C-Vertebral Artery1/RConn1 -- R- visco VA1/LConn1
  C-Radial Artery2/RConn1 -- R- Radial Artery2/LConn1
  R-Visco LEI1/LConn1 -- C- Left External Iliac1/RConn1
  R- visco RCCA1/RConn1 -- Electrical Reference108/LConn1
  C-Right Common Carotid A1/RConn1 -- R- visco RCCA1/LConn1
  R-Left Gastric Artery1/RConn1 -- L-Left Gastric Artery1/LConn1
  C- main Pulmonary Artery1/RConn1 -- R- Viscoelastic1/LConn1
  R-Visco RFA1/RConn1 -- Electrical Reference96/LConn1
  C- R Brachial1/RConn1 -- R-  R Brachial1/LConn1
  R-Visco Hepatic 1/LConn1 -- C- Hepatic Artery1/RConn1
  C- RSPV1/RConn1 -- Electrical Reference116/LConn1
  R- Right External Carotid1/RConn1 -- L-Right External Carotid1/LConn1
  C-axilary1/RConn1 -- R- visco axilary1/LConn1
  C- Anterior Tibial Artery1/RConn1 -- R-Visco AT1/LConn1
  R- visco axilary1/RConn1 -- Electrical Reference102/LConn1
  R- visco RIC1/RConn1 -- Electrical Reference112/LConn1
  R-Visco RCI1/LConn1 -- C-Right Common Iliac1/RConn1
  Resistor7/RConn1 -- Inductor4/LConn1
  C- Abdominal Aorta 2/RConn1 -- R-Viscoelastic AB2/LConn1
  R- Axillary1/RConn1 -- L-Axillary1/LConn1
  R- Superior Vena Cava3/RConn1 -- L- Superior Vena Cava1/LConn1
  R- visco RS1/RConn1 -- Electrical Reference111/LConn1
  R-Visco LR1/LConn1 -- C-  Left Renal Artery1/RConn1
  L-Inferior Mesentric1/LConn1 -- R- Inferior Mesentric1/RConn1
  R-Visco REI1/RConn1 -- Electrical Reference93/LConn1
  Electrical Reference120/LConn1 -- C- LSPV1/RConn1
  L-  Descending Aorta1/LConn1 -- R- Descending Aorta1/RConn1
  R-Visco RR1/RConn1 -- Electrical Reference86/LConn1
  Electrical Reference74/LConn1 -- R-Viscoelastic AB2/RConn1
  R-Visco LEI1/RConn1 -- Electrical Reference92/LConn1
  Voltage Sensor7/RConn1 -- PS-Simulink Converter7/LConn1
  R-Visco Left Gastric1/RConn1 -- Electrical Reference83/LConn1
  R-Visco IM1/RConn1 -- Electrical Reference89/LConn1
  Inductor3/LConn1 -- Resistor5/RConn1
  R- visco BrachiocephalicArtery1/RConn1 -- Electrical Reference107/LConn1
  L-Left Common Iliac1/LConn1 -- R-Left Common Iliac1/RConn1
  R- Right Gastric Artery1/RConn1 -- L- Right Gastric Artery1/LConn1
  Simulink-PS Converter2/RConn1 -- Controlled Voltage Source2/RConn1
  C-Ulnar Artery2/RConn1 -- R- Ulnar Artery2/LConn1
  Electrical Reference60/LConn1 -- Controlled Voltage Source2/RConn2
  R- visco REC1/RConn1 -- Electrical Reference113/LConn1
  R-Rdial Artery2/RConn1 -- L-Radial Artery2/LConn1
  Voltage Sensor5/RConn2 -- Electrical Reference73/LConn1
  C-BrachiocephalicArtery1/RConn1 -- R- visco BrachiocephalicArtery1/LConn1
  R-Visco LFA1/LConn1 -- C- Left Femoral Artery1/RConn1
  R- visco VA1/RConn1 -- Electrical Reference109/LConn1
  C-  L Anterior Tibial Artery1/RConn1 -- R- L Visco AT1/LConn1
  C- RPA1/RConn1 -- R-R Viscielastic1/LConn1
  Electrical Reference82/LConn1 -- R-Visco Right Gastric1/RConn1
  Resistor6/RConn1 -- Inductor5/LConn1
  R- Inferior Vena Cava1/LConn1 -- R- Superior Vena Cava5/LConn1
  R-Visco LR1/RConn1 -- Electrical Reference87/LConn1
  R-Ulnar Artery2/RConn1 -- L-Ulnar Artery2/LConn1
  R- Left Atrium1/RConn1 -- L- Left Atrium1/LConn1
  R-Visco RFA1/LConn1 -- C-Right Femoral Artery1/RConn1
  Simulink-PS Converter4/RConn1 -- Controlled Voltage Source4/RConn1
  R-Ulnar Artery3/RConn1 -- L-Ulnar Artery3/LConn1
  R- Ulnar Artery3/RConn1 -- Electrical Reference110/LConn1
  Electrical Reference77/LConn1 -- R- visco Left Subcalvin2/RConn1
  Electrical Reference103/LConn1 -- R- Radial Artery3/RConn1
  R- Right Internal Carotid1/RConn1 -- L-Right Internal Carotid1/LConn1
  R-Visco Splentic1/RConn1 -- Electrical Reference85/LConn1
  L-R Posterior Tibial Artery1/LConn1 -- R-R Posterior Tibial Artery1/RConn1
  R- Vertebral Artery1/RConn1 -- L-Vertebral Artery1/LConn1
  L- LPA1/LConn1 -- R- left Pulmonary Artery1/RConn1
  R-Visco Splentic1/LConn1 -- C- Splentic1/RConn1
  L-Right Femoral Artery1/LConn1 -- R-Right Femoral Artery1/RConn1
  C-BrachiocephalicArtery2/LConn1 -- L-BrachiocephalicArtery2/RConn1 -- L2/LConn1
  C-Ulnar Artery5/LConn1 -- R- R Brachial2/LConn1 -- L-Radial Artery5/RConn1 -- C-Radial Artery5/LConn1 -- L-Ulnar Artery5/RConn1
  R- Right Internal Carotid2/LConn1 -- R-Rdial Artery5/LConn1 -- Voltage Sensor11/LConn1 -- R-Ulnar Artery5/LConn1 -- R- Right External Carotid2/LConn1
  C- Splentic2/LConn1 -- C-  Left Renal Artery2/LConn1 -- L- Left Renal Artery2/RConn1 -- C- Right Renal Artery2/LConn1 -- L-Right Renal Artery2/RConn1 -- C- Superior Mesentric2/LConn1 -- L-Superior Mesentric2/RConn1 -- C- Inferior Mesentric2/LConn1 -- L-Inferior Mesentric2/RConn1 -- R-Left Common Iliac2/LConn1 -- R-Right Common Iliac2/LConn1 -- L-  Abdominal Aorta 3/RConn1 -- C- Abdominal Aorta 3/LConn1 -- C- Hepatic Artery2/LConn1 -- L-  Hepatic Artery2/RConn1 -- L- Right Gastric Artery2/RConn1 -- C- Right Gastric Artery2/LConn1 -- L-Left Gastric Artery2/RConn1 -- C- Left Gastric Artery2/LConn1 -- L-Splentic2/RConn1
  R- Superior Vena Cava7/LConn1 -- L-Radial Artery4/RConn1 -- C-Radial Artery4/LConn1 -- Voltage Sensor14/LConn1 -- C-Ulnar Artery4/LConn1 -- L-Ulnar Artery4/RConn1 -- C-Left Vertebral2/LConn1 -- L-Left Vertebral2/RConn1 -- R- Vertebral Artery2/LConn1
  R-RIPV2/LConn1 -- L- RPA2/RConn1 -- C- RPA2/LConn1 -- R- RSPV2/LConn1
  Solver Configuration2/RConn1 -- C- main Pulmonary Artery2/LConn1 -- L- main Pulmonary Artery2/RConn1 -- Voltage Sensor15/LConn1 -- R- left Pulmonary Artery2/LConn1 -- R-Right Pulmonary Artery2/LConn1
  Capacitor8/LConn1 -- R- Descending Aorta2/LConn1 -- L-2/LConn1 -- Inductor8/RConn1
  R- Axillary2/LConn1 -- L-Left Subcalvin3/RConn1 -- C-Left Subcalvin3/LConn1
  L- Right Ventricle2/RConn1 -- Pulmonary Valve2/LConn1 -- C- Right Ventricle2/LConn1
  R- Brachial2/LConn1 -- L-Axillary2/RConn1 -- C-Axilary2/LConn1
  L -LIPV2/RConn1 -- R- Left Atrium2/LConn1 -- C- RIPV2/LConn1 -- L- RIPV2/RConn1 -- L- RSPV2/RConn1 -- C- RSPV2/LConn1 -- L-LSPV2/RConn1 -- C- LSPV2/LConn1 -- C-LIPV2/LConn1
  C-Right Common Iliac2/LConn1 -- R-Right External Iliac2/LConn1 -- L-Right Common Iliac2/RConn1
  C- Left Atrium2/LConn1 -- Mitral Valve2/LConn1 -- L- Left Atrium2/RConn1
  L-Right External Carotid2/RConn1 -- L-Right Internal Carotid2/RConn1 -- C-Right Internal Carotid2/LConn1 -- R- Right Common Carotid A 2/LConn1 -- C-Right External Carotid2/LConn1
  L- Inferior Vena Cava2/RConn1 -- C- Inferior Vena Cava2/LConn1 -- R- Right Atrium2/LConn1 -- L- Superior Vena Cava2/RConn1 -- C- Superoir Vena Cava2/LConn1
  L-2/RConn1 -- R- Left Vertebral2/LConn1 -- R- Left Subcalvin 3/LConn1
  C-Vertebral Artery2/LConn1 -- C-Right Subclavin2/LConn1 -- L-Right Subclavin2/RConn1 -- R- BrachiocephalicArtery2/LConn1 -- L-Right Common Carotid A2/RConn1 -- C-Right Common Carotid A2/LConn1 -- L-Vertebral Artery2/RConn1
  Inductor7/RConn1 -- L2/RConn1 -- Resistor11/LConn1 -- Voltage Sensor13/LConn1 -- Capacitor7/LConn1
  L-Right Femoral Artery2/RConn1 -- R-L Posterior Tibial Artery2/LConn1 -- R-L Anterior Tibial Artery2/LConn1 -- C-Right Femoral Artery2/LConn1
  L- R Anterior Tibial Artery2/RConn1 -- R- Right Renal Artery2/LConn1 -- R- Left Renal Artery2/LConn1 -- R- Superior Mesentric2/LConn1 -- R- Superior Vena Cava8/RConn1 -- R- Right Gastric Artery2/LConn1 -- R- Hepatic Artery2/LConn1 -- R-Left Gastric Artery2/LConn1 -- R- Splentic2/LConn1 -- R- Inferior Mesentric2/LConn1 -- C- L Posterior Tibial Artery2/LConn1 -- L-L Posterior Tibial Artery2/RConn1 -- C-  L Anterior Tibial Artery2/LConn1 -- L- L Anterior Tibial Artery2/RConn1 -- C- Posterior Tibial Artery2/LConn1 -- L-R Posterior Tibial Artery2/RConn1 -- C- Anterior Tibial Artery2/LConn1
  C- Brachial2/LConn1 -- L- Brachial2/RConn1 -- R-Ulnar Artery4/LConn1 -- R-Rdial Artery4/LConn1
  R-LIPV2/LConn1 -- R- LSPV2/LConn1 -- L- LPA2/RConn1 -- C- LPA2/LConn1
  Mitral Valve2/RConn1 -- DC Voltage Source5/LConn1 -- Resistor10/LConn1
  R- Right Ventricle2/LConn1 -- DC Voltage Source6/LConn1 -- Tricuspid Valve2/RConn1
  L-Right External Iliac2/RConn1 -- R-Right Femoral Artery2/LConn1 -- C-Right External Iliac2/LConn1
  R-R Posterior Tibial Artery2/LConn1 -- C- Left Femoral Artery2/LConn1 -- L-Left Femoral Artery2/RConn1 -- R-R Anterior Tibial Artery2/LConn1
  C-axilary2/LConn1 -- R- Right Subclavin2/LConn1 -- L-axilary2/RConn1
  C- Left External Iliac2/LConn1 -- R-Left Femoral Artery2/LConn1 -- L-Left External Iliac2/RConn1
  L R Brachial2/RConn1 -- R- axilary2/LConn1 -- C- R Brachial2/LConn1
  C- Left Common Iliac2/LConn1 -- R-Left External Iliac2/LConn1 -- L-Left Common Iliac2/RConn1
  L- Right Atrium2/RConn1 -- Tricuspid Valve2/LConn1 -- C- Right Atrium2/LConn1
  L-  Descending Aorta2/RConn1 -- C- Descending Aorta2/LConn1 -- R-  Abdominal Aorta2/LConn1
  R-Visco Splentic2/LConn1 -- C- Splentic2/RConn1
  L- LPA2/LConn1 -- R- left Pulmonary Artery2/RConn1
  L-Right Femoral Artery2/LConn1 -- R-Right Femoral Artery2/RConn1
  L-R Posterior Tibial Artery2/LConn1 -- R-R Posterior Tibial Artery2/RConn1
  R- Right Internal Carotid2/RConn1 -- L-Right Internal Carotid2/LConn1
  Electrical Reference125/LConn1 -- R- Radial Artery5/RConn1
  Electrical Reference160/LConn1 -- R- visco Left Subcalvin3/RConn1
  R- Left Atrium2/RConn1 -- L- Left Atrium2/LConn1
  R-Ulnar Artery4/RConn1 -- L-Ulnar Artery4/LConn1
  R-Visco LR2/RConn1 -- Electrical Reference170/LConn1
  R- Inferior Vena Cava2/LConn1 -- R- Superior Vena Cava8/LConn1
  Resistor11/RConn1 -- Inductor8/LConn1
  C- RPA2/RConn1 -- R-R Viscielastic2/LConn1
  C-  L Anterior Tibial Artery2/RConn1 -- R- L Visco AT2/LConn1
  R- visco VA2/RConn1 -- Electrical Reference131/LConn1
  R-Visco LFA2/LConn1 -- C- Left Femoral Artery2/RConn1
  R-Visco Splentic2/RConn1 -- Electrical Reference168/LConn1
  Voltage Sensor12/RConn2 -- Electrical Reference156/LConn1
  R-Rdial Artery4/RConn1 -- L-Radial Artery4/LConn1
  C-Ulnar Artery4/RConn1 -- R- Ulnar Artery4/LConn1
  R- Right Gastric Artery2/RConn1 -- L- Right Gastric Artery2/LConn1
  L-Left Common Iliac2/LConn1 -- R-Left Common Iliac2/RConn1
  R-Visco IM2/RConn1 -- Electrical Reference172/LConn1
  Voltage Sensor13/RConn1 -- PS-Simulink Converter13/LConn1
  R-Visco LEI2/RConn1 -- Electrical Reference175/LConn1
  R-Visco RFA2/LConn1 -- C-Right Femoral Artery2/RConn1
  Electrical Reference157/LConn1 -- R-Viscoelastic AB3/RConn1
  R-Visco RR2/RConn1 -- Electrical Reference169/LConn1
  Electrical Reference142/LConn1 -- C- LSPV2/RConn1
  R-Visco REI2/RConn1 -- Electrical Reference176/LConn1
  L-Inferior Mesentric2/LConn1 -- R- Inferior Mesentric2/RConn1
  R- Axillary2/RConn1 -- L-Axillary2/LConn1
  Resistor12/RConn1 -- Inductor7/LConn1
  R-Visco RCI2/LConn1 -- C-Right Common Iliac2/RConn1
  R- visco RIC2/RConn1 -- Electrical Reference134/LConn1
  C- Anterior Tibial Artery2/RConn1 -- R-Visco AT2/LConn1
  C-axilary2/RConn1 -- R- visco axilary2/LConn1
  R- Right External Carotid2/RConn1 -- L-Right External Carotid2/LConn1
  R-Visco Hepatic 2/LConn1 -- C- Hepatic Artery2/RConn1
  C- R Brachial2/RConn1 -- R-  R Brachial2/LConn1
  R- visco axilary2/RConn1 -- Electrical Reference124/LConn1
  R-Visco RFA2/RConn1 -- Electrical Reference179/LConn1
  C- main Pulmonary Artery2/RConn1 -- R- Viscoelastic2/LConn1
  R-Left Gastric Artery2/RConn1 -- L-Left Gastric Artery2/LConn1
  C-Right Common Carotid A2/RConn1 -- R- visco RCCA2/LConn1
  R- visco RCCA2/RConn1 -- Electrical Reference130/LConn1
  R-Visco LEI2/LConn1 -- C- Left External Iliac2/RConn1
  C-Vertebral Artery2/RConn1 -- R- visco VA2/LConn1
  R- Viscoelastic2/RConn1 -- Electrical Reference148/LConn1
  Voltage Sensor15/RConn2 -- Electrical Reference150/LConn1
  R-Visco LFA2/RConn1 -- Electrical Reference177/LConn1
  Pulmonary Valve2/RConn1 -- R- main Pulmonary Artery2/LConn1
  C- Right Atrium2/RConn1 -- Electrical Reference153/LConn1
  R- visco Axilary2/RConn1 -- Electrical Reference162/LConn1
  Electrical Reference143/LConn1 -- C-LIPV2/RConn1
  C-Right Internal Carotid2/RConn1 -- R- visco RIC2/LConn1
  C- Abdominal Aorta 3/RConn1 -- R-Viscoelastic AB3/LConn1
  C-Right External Carotid2/RConn1 -- R- visco REC2/LConn1
  R-L Visco PT2/RConn1 -- Electrical Reference122/LConn1
  L-LSPV2/LConn1 -- R- LSPV2/RConn1
  R-Visco REI2/LConn1 -- C-Right External Iliac2/RConn1
  R- visco REC2/RConn1 -- Electrical Reference135/LConn1
  R- LPA2/RConn1 -- Electrical Reference128/LConn1
  Simulink-PS Converter5/RConn1 -- Controlled Voltage Source5/RConn1
  Electrical Reference127/LConn1 -- Resistor13/RConn1
  R- Right Atrium2/RConn1 -- L- Right Atrium2/LConn1
  L-L Posterior Tibial Artery2/LConn1 -- R-L Posterior Tibial Artery2/RConn1
  C-Right Subclavin2/RConn1 -- R- visco RS2/LConn1
  R-Visco RCI2/RConn1 -- Electrical Reference174/LConn1
  R-Visco Right Gastric2/LConn1 -- C- Right Gastric Artery2/RConn1
  R-Visco PT2/RConn1 -- Electrical Reference181/LConn1
  R- Left Vertebral2/RConn1 -- L-Left Vertebral2/LConn1
  C-Left Subcalvin3/RConn1 -- R- visco Left Subcalvin3/LConn1
  L- main Pulmonary Artery2/LConn1 -- R- main Pulmonary Artery2/RConn1
  R-RIPV2/RConn1 -- L- RIPV2/LConn1
  C- RSPV2/RConn1 -- Electrical Reference138/LConn1
  C-Left Vertebral2/RConn1 -- R- visco Left Vertebral2/LConn1
  L- RSPV2/LConn1 -- R- RSPV2/RConn1
  R- Ulnar Artery4/RConn1 -- Electrical Reference140/LConn1
  C-Ulnar Artery5/RConn1 -- R- Ulnar Artery5/LConn1
  Electrical Reference151/LConn1 -- Resistor14/RConn1
  Controlled Voltage Source6/LConn1 -- DC Voltage Source6/RConn1
  R-Visco LCI2/RConn1 -- Electrical Reference173/LConn1
  R- visco BrachiocephalicArtery2/RConn1 -- Electrical Reference129/LConn1
  Electrical Reference164/LConn1 -- R-Visco Hepatic 2/RConn1
  R-Visco LCI2/LConn1 -- C- Left Common Iliac2/RConn1
  Simulink-PS Converter6/RConn1 -- Controlled Voltage Source6/RConn1
  Resistor14/LConn1 -- Capacitor7/RConn1
  R-Visco RR2/LConn1 -- C- Right Renal Artery2/RConn1
  Voltage Sensor11/RConn2 -- Electrical Reference123/LConn1
  R- Superior Vena Cava6/RConn1 -- L- Superior Vena Cava2/LConn1
  L-Right Common Iliac2/LConn1 -- R-Right Common Iliac2/RConn1
  R-  R Brachial2/RConn1 -- Electrical Reference126/LConn1
  R- BrachiocephalicArtery2/RConn1 -- L-BrachiocephalicArtery2/LConn1
  R- Right Renal Artery2/RConn1 -- L-Right Renal Artery2/LConn1
  C-Axilary2/RConn1 -- R- visco Axilary2/LConn1
  Inductor6/LConn1 -- Resistor10/RConn1
  C- Left Atrium2/RConn1 -- Electrical Reference178/LConn1
  C- Brachial2/RConn1 -- R- visco  Brachial2/LConn1
  Electrical Reference149/LConn1 -- R- Radial Artery4/RConn1
  C- Inferior Mesentric2/RConn1 -- R-Visco IM2/LConn1
  C-Radial Artery5/RConn1 -- R- Radial Artery5/LConn1
  L-Right External Iliac2/LConn1 -- R-Right External Iliac2/RConn1
  Capacitor6/RConn1 -- Electrical Reference144/LConn1
  L-axilary2/LConn1 -- R- axilary2/RConn1
  Electrical Reference171/LConn1 -- R-Visco SM2/RConn1
  R-R Anterior Tibial Artery2/RConn1 -- L- R Anterior Tibial Artery2/LConn1
  R- Superior Mesentric2/RConn1 -- L-Superior Mesentric2/LConn1
  Electrical Reference158/LConn1 -- R-Viscoelastic DA2/RConn1
  Electrical Reference159/LConn1 -- C- Inferior Vena Cava2/RConn1
  Electrical Reference147/LConn1 -- C- Right Ventricle2/RConn1
  Voltage Sensor15/RConn1 -- PS-Simulink Converter15/LConn1
  R-LIPV2/RConn1 -- L -LIPV2/LConn1
  L- RPA2/LConn1 -- R-Right Pulmonary Artery2/RConn1
  L- Inferior Vena Cava2/LConn1 -- R- Inferior Vena Cava2/RConn1
  PS-Simulink Converter14/LConn1 -- Voltage Sensor14/RConn1
  R- Left Subcalvin 3/RConn1 -- L-Left Subcalvin3/LConn1
  Electrical Reference145/LConn1 -- Controlled Voltage Source5/RConn2
  L- Right Ventricle2/LConn1 -- R- Right Ventricle2/RConn1
  L-  Descending Aorta2/LConn1 -- R- Descending Aorta2/RConn1
  L-  Abdominal Aorta 3/LConn1 -- R-  Abdominal Aorta2/RConn1
  R- Left Renal Artery2/RConn1 -- L- Left Renal Artery2/LConn1
  R-Visco Left Gastric2/RConn1 -- Electrical Reference166/LConn1
  Voltage Sensor13/RConn2 -- Electrical Reference155/LConn1
  C- LPA2/RConn1 -- R- LPA2/LConn1
  C-Radial Artery4/RConn1 -- R- Radial Artery4/LConn1
  Voltage Sensor14/RConn2 -- Electrical Reference152/LConn1
  R- Right Common Carotid A 2/RConn1 -- L-Right Common Carotid A2/LConn1
  R-Visco LR2/LConn1 -- C-  Left Renal Artery2/RConn1
  L R Brachial2/LConn1 -- R- R Brachial2/RConn1
  R-Rdial Artery5/RConn1 -- L-Radial Artery5/LConn1
  C- RIPV2/RConn1 -- Electrical Reference141/LConn1
  R- visco RS2/RConn1 -- Electrical Reference133/LConn1
  R- visco  Brachial2/RConn1 -- Electrical Reference163/LConn1
  R-Visco SM2/LConn1 -- C- Superior Mesentric2/RConn1
  DC Voltage Source5/RConn1 -- Controlled Voltage Source5/LConn1
  Voltage Sensor11/RConn1 -- PS-Simulink Converter11/LConn1
  Voltage Sensor12/LConn1 -- Mitral Valve4/LConn1 -- Inductor6/RConn1 -- Capacitor6/LConn1
  C- Superoir Vena Cava2/RConn1 -- Electrical Reference154/LConn1
  R-Left Femoral Artery2/RConn1 -- L-Left Femoral Artery2/LConn1
  R- Splentic2/RConn1 -- L-Splentic2/LConn1
  C- Posterior Tibial Artery2/RConn1 -- R-Visco PT2/LConn1
  C- Descending Aorta2/RConn1 -- R-Viscoelastic DA2/LConn1
  R-L Anterior Tibial Artery2/RConn1 -- L- L Anterior Tibial Artery2/LConn1
  R-Visco AT2/RConn1 -- Electrical Reference180/LConn1
  Resistor13/LConn1 -- Capacitor8/RConn1
  R- Superior Vena Cava6/LConn1 -- R- Superior Vena Cava7/RConn1
  R-R Viscielastic2/RConn1 -- Electrical Reference146/LConn1
  R- L Visco AT2/RConn1 -- Electrical Reference182/LConn1
  R-Visco Left Gastric2/LConn1 -- C- Left Gastric Artery2/RConn1
  Voltage Sensor12/RConn1 -- PS-Simulink Converter12/LConn1
  R- Ulnar Artery5/RConn1 -- Electrical Reference132/LConn1
  R- Brachial2/RConn1 -- L- Brachial2/LConn1
  R-Ulnar Artery5/RConn1 -- L-Ulnar Artery5/LConn1
  R-Left External Iliac2/RConn1 -- L-Left External Iliac2/LConn1
  R- Hepatic Artery2/RConn1 -- L-  Hepatic Artery2/LConn1
  R- visco Left Vertebral2/RConn1 -- Electrical Reference139/LConn1
  Electrical Reference165/LConn1 -- R-Visco Right Gastric2/RConn1
  C- L Posterior Tibial Artery2/RConn1 -- R-L Visco PT2/LConn1
  R- Right Subclavin2/RConn1 -- L-Right Subclavin2/LConn1
  R- Vertebral Artery2/RConn1 -- L-Vertebral Artery2/LConn1
  C-BrachiocephalicArtery2/RConn1 -- R- visco BrachiocephalicArtery2/LConn1
  C- Left External Iliac3/LConn1 -- R-Left Femoral Artery3/LConn1 -- L-Left External Iliac3/RConn1
  Resistor16/LConn1 -- L3/RConn1 -- Voltage Sensor18/LConn1 -- Capacitor10/LConn1 -- Inductor10/RConn1
  C- RPA3/LConn1 -- L- RPA3/RConn1 -- R- RSPV3/LConn1 -- R-RIPV3/LConn1
  C- Right Gastric Artery3/LConn1 -- L- Right Gastric Artery3/RConn1 -- C- Hepatic Artery3/LConn1 -- L-  Hepatic Artery3/RConn1 -- L-Left Gastric Artery3/RConn1 -- C- Left Gastric Artery3/LConn1 -- L-Splentic3/RConn1 -- C- Splentic3/LConn1 -- L-  Abdominal Aorta 4/RConn1 -- C- Abdominal Aorta 4/LConn1 -- C- Superior Mesentric3/LConn1 -- L-Superior Mesentric3/RConn1 -- C- Right Renal Artery3/LConn1 -- L-Right Renal Artery3/RConn1 -- C-  Left Renal Artery3/LConn1 -- L- Left Renal Artery3/RConn1 -- R-Left Common Iliac3/LConn1 -- R-Right Common Iliac3/LConn1 -- C- Inferior Mesentric3/LConn1 -- L-Inferior Mesentric3/RConn1
  Voltage Sensor19/LConn1 -- L-Radial Artery6/RConn1 -- C-Radial Artery6/LConn1 -- C-Ulnar Artery6/LConn1 -- L-Ulnar Artery6/RConn1 -- C-Left Vertebral3/LConn1 -- L-Left Vertebral3/RConn1 -- R- Vertebral Artery3/LConn1 -- R- Superior Vena Cava10/LConn1
  L -LIPV3/RConn1 -- C-LIPV3/LConn1 -- L-LSPV3/RConn1 -- C- LSPV3/LConn1 -- R- Left Atrium3/LConn1 -- L- RSPV3/RConn1 -- C- RSPV3/LConn1 -- C- RIPV3/LConn1 -- L- RIPV3/RConn1
